simulink model "SWC_HALOUT_type"  (R2021b)
settings: Solver=FixedStepDiscrete  StartTime=0.0  StopTime=10.0  FixedStep=0.005  RelTol=1e-3
undefined symbols (not defined in the file): DIDLen_APPD, DIDLen_APPE, DIDLen_APPPedalZP, DIDLen_APSFunConfig, DIDLen_AutoLock, DIDLen_AutoWipHSpdEN, DIDLen_CALID, DIDLen_CDEODT, DIDLen_CLRDIST, DIDLen_DKCBLESta, DIDLen_DKCKey, DIDLen_DKCSta, DIDLen_DoorNFCAnchorSta, DIDLen_DRLDis, DIDLen_DynoMode, DIDLen_ECUNAME, DIDLen_FDDKCCoordXY, DIDLen_FMHTimer, DIDLen_LFLowPresThre, DIDLen_LFSensorID, DIDLen_LIDAAnchorSta, DIDLen_LRLowPresThre, DIDLen_LRSensorID, DIDLen_MILDIST, DIDLen_NUMPSATRIPSFLTMEMCLR, DIDLen_NVMPedalZP, DIDLen_OBDReq, DIDLen_ODOMETER, DIDLen_PKE, DIDLen_ProtocolId, DIDLen_PSA, DIDLen_QTYPSATRIPS, DIDLen_RFLowPresThre, DIDLen_RFSensorID, DIDLen_RRLowPresThre, DIDLen_RRSensorID, DIDLen_RUNTM, DIDLen_SensorMode, DIDLen_TestGroup, DIDLen_TireSize, DIDLen_TPMSLearnSta, DIDLen_TurnLampFLThreCurr, DIDLen_TurnLampFRThreCurr, DIDLen_TurnLampRLThreCurr, DIDLen_TurnLampRRThreCurr, DIDLen_UIDSta, DIDLen_USSConfig, DIDLen_UWBAnchorSta, DIDLen_VIN, DIDLen_VSS, DIDLen_WhlPres, DIDLen_WhlSensorBattSta, DIDLen_WhlTmp, DIDLen_WipRLSCmdCutFilter, DIDLen_WipRLSCmdHoldFilter, DIDLen_XWDMode, DIDNum_APPD, DIDNum_APPE, DIDNum_APPPedalZP, DIDNum_APSFunConfig ... (+504)
libraries: simulink x893, FVT_lib x320, hdlsllib x6, hcu_lib x5, halout x1
(part 10 of 11)

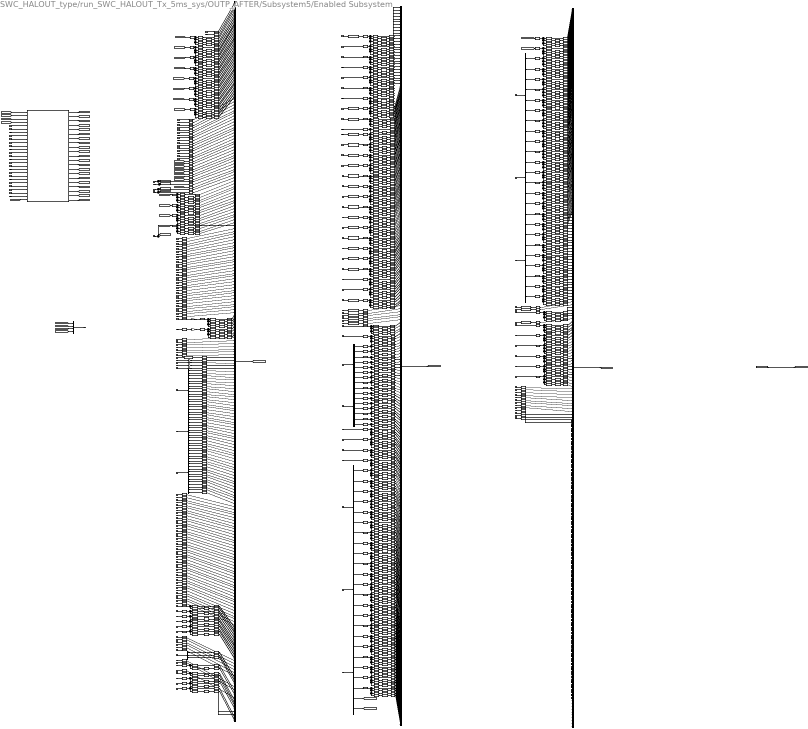
== system SWC_HALOUT_type/run_SWC_HALOUT_Tx_5ms_sys/OUTP_AFTER/Subsystem5/Enabled Subsystem ==
  VOUTP_AntitheftSta_enum : Inport
  VOUTP_DrivetrainSelect_enum : Inport  Port=2
  VOUTP_WriteChkLFID_raw : Inport  Port=3
  VOUTP_WriteChkRFID_raw : Inport  Port=4
  VOUTP_WriteChkLRID_raw : Inport  Port=5
  VOUTP_WriteChkRRID_raw : Inport  Port=6
  VOUTP_WriteChkfinLFID_raw : Inport  Port=7
  VOUTP_WriteChkfinRFID_raw : Inport  Port=8
  VOUTP_WriteChkfinLRID_raw : Inport  Port=9
  VOUTP_WriteChkfinRRID_raw : Inport  Port=10
  VOUTP_LFSensorFail_flg : Inport  Port=11
  VOUTP_RFSensorFail_flg : Inport  Port=12
  VOUTP_LRSensorFail_flg : Inport  Port=13
  VOUTP_RRSensorFail_flg : Inport  Port=14
  VOUTP_LFWheelPSW_raw8 : Inport  Port=15
  VOUTP_RFWheelPSW_raw8 : Inport  Port=16
  VOUTP_LRWheelPSW_raw8 : Inport  Port=17
  VOUTP_RRWheelPSW_raw8 : Inport  Port=18
  VOUTP_LFPindi_enum : Inport  Port=19
  VOUTP_RFPindi_enum : Inport  Port=20
  VOUTP_LRPindi_enum : Inport  Port=21
  VOUTP_RRPindi_enum : Inport  Port=22
  VOUTP_LFP20_raw8 : Inport  Port=23
  VOUTP_RFP20_raw8 : Inport  Port=24
  VOUTP_LRP20_raw8 : Inport  Port=25
  VOUTP_RRP20_raw8 : Inport  Port=26
  VOUTP_LFWheelPress_raw8 : Inport  Port=27
  VOUTP_RFWheelPress_raw8 : Inport  Port=28
  VOUTP_LRWheelPress_raw8 : Inport  Port=29
  VOUTP_RRWheelPress_raw8 : Inport  Port=30
  VOUTP_LFWheelTemp_C : Inport  Port=31
  VOUTP_RFWheelTemp_C : Inport  Port=32
  VOUTP_LRWheelTemp_C : Inport  Port=33
  VOUTP_RRWheelTemp_C : Inport  Port=34
  VOUTP_Flashchkdatavalid_enum : Inport  Port=35
  VOUTP_Flashdatavalid_enum : Inport  Port=36
  VOUTP_unlearnSfali_flg : Inport  Port=37
  VOUTP_unlearnSfailvalid_enum : Inport  Port=38
  VOUTP_Prepresstempvalid_enum : Inport  Port=39
  VOUTP_FlashS1ID_raw : Inport  Port=40
  VOUTP_FlashS2ID_raw : Inport  Port=41
  VOUTP_FlashS3ID_raw : Inport  Port=42
  VOUTP_FlashS41ID_raw : Inport  Port=43
  VOUTP_FlashIDvalid_enum : Inport  Port=44
  VOUTP_ACModeMem_enum : Inport  Port=45
  VOUTP_Face_flg : Inport  Port=46
  VOUTP_Foot_flg : Inport  Port=47
  VOUTP_Frost_flg : Inport  Port=48
  VOUTP_FaceM_flg : Inport  Port=49
  VOUTP_FootM_flg : Inport  Port=50
  VOUTP_CCUSyncSts_flg : Inport  Port=51
  VOUTP_ACForceOFF_flg : Inport  Port=52
  VOUTP_sigRecircSt_flg : Inport  Port=53
  VOUTP_RecAutoFlg_flg : Inport  Port=54
  VOUTP_AirIntenZone1M_enum : Inport  Port=55
  VOUTP_fdefog_flg : Inport  Port=56
  VOUTP_sigSetTempZon1St_C : Inport  Port=57
  VOUTP_sigSetTempZon2StM_C : Inport  Port=58
  VOUT_CountAlarm_enum : Inport  Port=59
  VOUTP_MFSWTri_flg : Inport  Port=60
  VOUTP_MirrorFlodPos_flg : Inport  Port=61
  VOUTP_FuelDoorPos_flg : Inport  Port=62
  VOUTP_LockSetting_flg : Inport  Port=63
  VOUTP_MFRDNBrightReq_pct : Inport  Port=64
  VOUTP_RoomLampMode_flg : Inport  Port=65
  VOUTP_WiperFixMode_flg : Inport  Port=66
  VOUTP_IVIPTGUSStaSW_flg : Inport  Port=67
  VOUTP_EAPS1MIN_pct : Inport  Port=68
  VOUTP_EAPS2MIN_pct : Inport  Port=69
  VOUTP_HoodSW_flg : Inport  Port=70
  VOUTP_TailgateSW_flg : Inport  Port=71
  VOUTP_CTDLockSW_flg : Inport  Port=72
  VOUTP_TailgateHDSW_flg : Inport  Port=73
  VOUTP_APMDoorControlSta_flg : Inport  Port=74
  VOUTP_fUnlockSingle_flg : Inport  Port=75
  VOUTP_SaveRegenMode_enum : Inport  Port=76
  VOUTP_AmbFunENFlash_enum : Inport  Port=77
  VOUTP_AmbWelENFlash_enum : Inport  Port=78
  VOUTP_AmbDimENFlash_enum : Inport  Port=79
  VOUTP_AmbLinkDriStaFlash_enum : Inport  Port=80
  VOUTP_AmbPwrWarnENFlash_enum : Inport  Port=81
  VOUTP_AmbODAENFlash_enum : Inport  Port=82
  VOUTP_AmbColorSta1_enum : Inport  Port=83
  VOUTP_AmbColorSta2_enum : Inport  Port=84
  VOUTP_AmbColorSta3_enum : Inport  Port=85
  VOUTP_AmbColorSta4_enum : Inport  Port=86
  VOUTP_AmbColorSta5_enum : Inport  Port=87
  VOUTP_AmbColorSta7_enum : Inport  Port=88
  VOUTP_AmbBrightnessSta1_enum : Inport  Port=89
  VOUTP_AmbBrightnessSta2_enum : Inport  Port=90
  VOUTP_AmbBrightnessSta3_enum : Inport  Port=91
  VOUTP_AmbBrightnessSta4_enum : Inport  Port=92
  VOUTP_AmbBrightnessSta5_enum : Inport  Port=93
  VOUTP_AmbBrightnessSta7_enum : Inport  Port=94
  VOUTP_TurnSwTimeSetSta123_enum : Inport  Port=95
  VOUTP_TurnSwTimeSetSta457_enum : Inport  Port=96
  VOUTP_FDCTHCAirIntZ3Sta_enum : Inport  Port=97
  VOUTP_FDCTHCREVentModeSta_enum : Inport  Port=98
  VOUTP_FDCTHCLEVentModeSta_enum : Inport  Port=99
  VOUTP_FDCTHCLEVentZSta_enum : Inport  Port=100
  VOUTP_FDCTHCCLEVentZSta_enum : Inport  Port=101
  VOUTP_FDCTHCREVentZSta_enum : Inport  Port=102
  VOUTP_FDCTHCCREVentZSta_enum : Inport  Port=103
  VOUTP_LVentEN_flg : Inport  Port=104
  VOUTP_FDCTHCLEVentYSta_enum : Inport  Port=105
  VOUTP_CLVentEN_flg : Inport  Port=106
  VOUTP_FDCTHCCLEVentYSta_enum : Inport  Port=107
  VOUTP_RVentEN_flg : Inport  Port=108
  VOUTP_FDCTHCREVentYSta_enum : Inport  Port=109
  VOUTP_CRVentEN_flg : Inport  Port=110
  VOUTP_FDCTHCCREVentYSta_enum : Inport  Port=111
  VOUTP_FDCFGSAirIntSta_enum : Inport  Port=112
  VOUTP_FDCFGSChSta_enum : Inport  Port=113
  VOUTP_FDCFGSIONSWSta_flg : Inport  Port=114
  VOUTP_WalkOutLkENFunSta_flg : Inport  Port=115
  VOUTP_WalkInUnLkENFunSta_flg : Inport  Port=116
  VOUTP_FollowMeENFunSta_flg : Inport  Port=117
  VOUTP_PTGUserHeight1_cnt : Inport  Port=118
  VOUTP_PTGUserHeight2_cnt : Inport  Port=119
  VOUTP_PTGUserHeight3_cnt : Inport  Port=120
  VOUTP_PTGUserHeight4_cnt : Inport  Port=121
  VOUTP_PTGUserHeight5_cnt : Inport  Port=122
  VOUTP_PTGUserHeight7_cnt : Inport  Port=123
  VOUTP_PTGOpenHeight12_enum : Inport  Port=124
  VOUTP_PTGOpenHeight34_enum : Inport  Port=125
  VOUTP_PTGOpenHeight57_enum : Inport  Port=126
  VOUTP_ACCLevelMem12_enum : Inport  Port=127
  VOUTP_ACCLevelMem34_enum : Inport  Port=128
  VOUTP_ACCLevelMem57_enum : Inport  Port=129
  VOUTP_AutoLockMem_enum : Inport  Port=130
  VOUTP_AutoUnlockMem_enum : Inport  Port=131
  VOUTP_MILDIST_km : Inport  Port=132
  VOUTP_CLRDIST_km : Inport  Port=133
  VOUTP_WARMUPS_cnt : Inport  Port=134
  VOUTP_MILTIME_min : Inport  Port=135
  VOUTP_CLRTIME_min : Inport  Port=136
  VOUTP_NUMPSATRIPSFLTMEMCLR_cnt : Inport  Port=137
  VOUTP_PSAR_sec : Inport  Port=138
  VOUTP_PSAL_sec : Inport  Port=139
  VOUTP_IPSAR_sec : Inport  Port=140
  VOUTP_IPSAL_sec : Inport  Port=141
  VOUTP_CPSAR_sec : Inport  Port=142
  VOUTP_CPSAL_sec : Inport  Port=143
  VOUTP_HVBNAH_Ahr : Inport  Port=144
  VOUTP_IGNCNTR_cnt : Inport  Port=145
  VOUTP_TNBCPSAR_Ahr : Inport  Port=146
  VOUTP_TNBCPSAL_Ahr : Inport  Port=147
  VOUTP_TNECPSAR_kWh : Inport  Port=148
  VOUTP_TNECPSAL_kWh : Inport  Port=149
  VOUTP_TEBPSAR_kWh : Inport  Port=150
  VOUTP_TEBPSAL_kWh : Inport  Port=151
  VOUTP_TGEOVCR_kWh : Inport  Port=152
  VOUTP_TGEOVCL_kWh : Inport  Port=153
  VOUTP_GECHGOVCDCR_kWh : Inport  Port=154
  VOUTP_GECHGOVCDCL_kWh : Inport  Port=155
  VOUTP_GECHGOVCACR_kWh : Inport  Port=156
  VOUTP_GECHGOVCACL_kWh : Inport  Port=157
  VOUTP_RESSV2XENNONPSAR_kWh : Inport  Port=158
  VOUTP_RESSV2XENNONPSAL_kWh : Inport  Port=159
  VOUTP_PKERNumerator_kphsqr : Inport  Port=160
  VOUTP_PKELNumerator_kphsqr : Inport  Port=161
  VOUTP_ODOMETER_km : Inport  Port=162
  VOUTP_ResetCDEODTR_km : Inport  Port=163
  VOUTP_AvgBattTempPSAR_C : Inport  Port=164
  VOUTP_AvgBattTempPSAL_C : Inport  Port=165
  VOUTP_AvgBattTempOVCR_C : Inport  Port=166
  VOUTP_AvgBattTempOVCL_C : Inport  Port=167
  VOUTP_AvgBattTempOFFR_C : Inport  Port=168
  VOUTP_AvgBattTempOFFL_C : Inport  Port=169
  VOUTP_HVBNE_kWh : Inport  Port=170
  VOUTP_QTYPSATRIPSR_cnt : Inport  Port=171
  VOUTP_QTYPSATRIPSL_cnt : Inport  Port=172
  VOUTP_RESSCNTDODRNGR_cnt : Inport  Port=173
  VOUTP_ETMBTOER_kWh : Inport  Port=174
  VOUTP_ETMBTOEL_kWh : Inport  Port=175
  VOUTP_RESSCNTDODRNGL_cnt : Inport  Port=176
  VOUTP_ETMATOER_kWh : Inport  Port=177
  VOUTP_ETMATOEL_kWh : Inport  Port=178
  VOUTP_RESSTIMESOCPSARNGR_s : Inport  Port=179
  VOUTP_RESSTIMESOCPSARNGL_s : Inport  Port=180
  VOUTP_RESSTIMESOCCHGRNGR_s : Inport  Port=181
  VOUTP_RESSTIMESOCOFFRNGL_s : Inport  Port=182
  VOUTP_MAXBATTEMPL_C : Inport  Port=183
  VOUTP_MINBATTEMPL_C : Inport  Port=184
  VOUTP_RESSTIMESOCCHGRNGL_s : Inport  Port=185
  VOUTP_RESSTIMESOCOFFRNGR_s : Inport  Port=186
  VOUTP_AVGBATTEMPL_sec : Inport  Port=187
  VOUTP_AVGBATTEMPL_C : Inport  Port=188
  VOUTP_BattTempPSAR_sec : Inport  Port=189
  VOUTP_BattTempPSAL_sec : Inport  Port=190
  VOUTP_OVCR_sec : Inport  Port=191
  VOUTP_OVCL_sec : Inport  Port=192
  VOUTP_OFFR_sec : Inport  Port=193
  VOUTP_OFFL_sec : Inport  Port=194
  VOUTP_HMIKey1FuncSta_enum : Inport  Port=195
  VOUTP_HMIKey2FuncSta_enum : Inport  Port=196
  VOUTP_HMIKey3FuncSta_enum : Inport  Port=197
  VOUTP_HMIKey4FuncSta_enum : Inport  Port=198
  VOUTP_HMIKey5FuncSta_enum : Inport  Port=199
  VOUTP_HMIKey6FuncSta_enum : Inport  Port=200
  VOUTP_HMIKey7FuncSta_enum : Inport  Port=201
  VOUTP_HMIKey8FuncSta_enum : Inport  Port=202
  VOUTP_AutoWipHSpdENSta_flg : Inport  Port=203
  VOUTP_ModelVersion_raw : Inport  Port=204
  VOUTP_ModelVersionChksum_raw : Inport  Port=205
  VOUTP_DIDModelVersion_raw : Inport  Port=206
  VOUTP_DIDModelVersionChksum_raw : Inport  Port=207
  BHAL_SYS_outputs : Inport  Port=208
  VHAL_RandomnumberY_raw1 : Inport  Port=209
  VHAL_RandomnumberY_raw2 : Inport  Port=210
  VHAL_RandomnumberY_raw3 : Inport  Port=211
  VHAL_RandomnumberY_raw4 : Inport  Port=212
  VHAL_RandomnumberY_raw5 : Inport  Port=213
  VHAL_RandomnumberY_raw6 : Inport  Port=214
  VHAL_RandomnumberY_raw7 : Inport  Port=215
  VHAL_RandomnumberY_raw8 : Inport  Port=216
  VHAL_funAuto_flg : Inport  Port=217
  VHAL_DiagDRLOFF_flg : Inport  Port=218
  VHAL_DiagFMHT_s : Inport  Port=219
  VHAL_DiagFLTC_mA : Inport  Port=220
  VHAL_DiagFRTC_mA : Inport  Port=221
  VHAL_DiagRLTC_mA : Inport  Port=222
  VHAL_DiagRRTC_mA : Inport  Port=223
  VHAL_USSConfig_raw8 : Inport  Port=224
  VHAL_TireSize_raw8 : Inport  Port=225
  VHAL_APSFunConfig_raw8 : Inport  Port=226
  BHAL_DIDGetData_raw : Inport  Port=227
  Bitwise AND{,4,8,14,16,22,26,30,32,36,40,44,48,52,56,58,60,62,64,66,68,70,72,74,76,80,82,86,90,94,98,102,106,110,114,116,120,124,128,132,136,140,144,148,152,156,160,164,168,172,176,180,184,188,192,194,196,198,200,202,204,206,208,210,212,214,216,218,220,222,224,228,232,236,240,244,248,252,256,260,264,268,272,276,280,284,288,292,296,300,304,308,312,316,320,324,328,332,336,340,344,348,352,356,360,364,368,372,376,380,384,388,392,396,400,404,408,412,416,420,424,428,432,436,440,444,448,452,456} (129 alike) : simulink/Logic and Bit Operations/Bitwise Operator  logicop=AND  UseBitMask=on  BitMask=bin2dec('00000000000000000000000011111111')  BitMaskRealWorld=Stored Integer
  Bitwise AND{1,5,9,15,17,23,27,31,33,37,41,45,49,53,57,59,61,63,65,67,69,71,73,75,77,81,83,87,91,95,99,103,107,111,115,117,121,125,129,133,137,141,145,149,153,157,161,165,169,173,177,181,185,189,193,195,197,199,201,203,205,207,209,211,213,215,217,219,221,223,225,229,233,237,241,245,249,253,257,261,265,269,273,277,281,285,289,293,297,301,305,309,313,317,321,325,329,333,337,341,345,349,353,357,361,365,369,373,377,381,385,389,393,397,401,405,409,413,417,421,425,429,433,437,441,445,449,453,457} (129 alike) : simulink/Logic and Bit Operations/Bitwise Operator  logicop=AND  UseBitMask=on  BitMask=bin2dec('00000000000000001111111100000000')  BitMaskRealWorld=Stored Integer
  Bitwise AND{2,6,10,12,18,20,24,28,34,38,42,46,50,54,78,84,88,92,96,100,104,108,112,118,122,126,130,134,138,142,146,150,154,158,162,166,170,174,178,182,186,190,226,230,234,238,242,246,250,254,258,262,266,270,274,278,282,286,290,294,298,302,306,310,314,318,322,326,330,334,338,342,346,350,354,358,362,366,370,374,378,382,386,390,394,398,402,406,410,414,418,422,426,430,434,438,442,446,450,454,458} (101 alike) : simulink/Logic and Bit Operations/Bitwise Operator  logicop=AND  UseBitMask=on  BitMask=bin2dec('00000000111111110000000000000000')  BitMaskRealWorld=Stored Integer
  Bitwise AND{3,7,11,13,19,21,25,29,35,39,43,47,51,55,79,85,89,93,97,101,105,109,113,119,123,127,131,135,139,143,147,151,155,159,163,167,171,175,179,183,187,191,227,231,235,239,243,247,251,255,259,263,267,271,275,279,283,287,291,295,299,303,307,311,315,319,323,327,331,335,339,343,347,351,355,359,363,367,371,375,379,383,387,391,395,399,403,407,411,415,419,423,427,431,435,439,443,447,451,455,459} (101 alike) : simulink/Logic and Bit Operations/Bitwise Operator  logicop=AND  UseBitMask=on  BitMask=bin2dec('11111111000000000000000000000000')  BitMaskRealWorld=Stored Integer
  Bus Selector2 : BusSelector  OutputSignals=VHAL_AutoWipHSpdEN_raw,VHAL_WipRLSCmdHoldFilter_raw,VHAL_WipRLSCmdCutFilter_raw
  Constant : Constant  Value=zeros(256,1)  OutDataTypeStr=uint8
  Data Type Conversion{,1,5..13,15..18,20..23,25..27,29..32,34..37,39..40,42..106,108..111,113..116,118..121,123..126,128..130,132..235,237..239,241..242,244..245,247..248,250..251,253..265,267..269,271..272,274..275,277..278,280..283,285..286,288..291,293..296,298..301,303..306,308..311,313..316,318..321,323..326,328..329,331..334,336..339,341..344,346..349,351..354,356..359,361..364,366..369,371..374,376..379,381..384,386..389,391..394,396..399,401..404,406..415,417..420,422..425,427..430,432..433,435..436,438..439,441..442,444..445,447..448,450..451,453..454,456..457,459..460,462..463,465..466,468..469,471..472,474..475,477..478,480..483,485..488,490..493,495..498,500..503,505..508,510..513,515..518,520..523,525..528,530..533,535..538,540..543,545..548,550..553,555..558,560..563,565..568,570..573,575..578,580..583,585..588,590..593,595..598,600..603,605..608,610..613,615..618,620..623,625..628,630..633,635..638,640..643,645..648,650..653,655..658,660..663,665..668,670..673,675..678,680..683,685..688,690..693,695..698,700..703,705..708,710..713,715..718,720..723,725..728,730..733,735..740,742..746,748..751,753..756,758..761,763..766,768..771,773..789} (659 alike) : DataTypeConversion  OutDataTypeStr=uint8
  Data Type Conversion{4,14,19,24,28,33,38,41,107,112,117,122,127,131,279,287,292,297,302,307,312,317,322,330,335,340,345,350,355,360,365,370,375,380,385,390,395,400,405,416,421,426,479,484,489,494,499,504,509,514,519,524,529,534,539,544,549,554,559,564,569,574,579,584,589,594,599,604,609,614,619,624,629,634,639,644,649,654,659,664,669,674,679,684,689,694,699,704,709,714,719,724,729,734,741,747,752,757,762,767,772} (101 alike) : DataTypeConversion  OutDataTypeStr=uint32
  Data Type Conversion2 : DataTypeConversion  OutDataTypeStr=single
  Data Type Conversion{236,240,243,246,249,252,266,270,273,276,284,327,431,434,437,440,443,446,449,452,455,458,461,464,467,470,473,476} (28 alike) : DataTypeConversion  OutDataTypeStr=uint16
  Data Type Conversion3 : DataTypeConversion  OutDataTypeStr=single
  Demux : Demux  Outputs=16
  Demux1 : Demux  Outputs=16
  Demux{3..10} (8 alike) : Demux  Outputs=8
  Demux2 : Demux  Outputs=16
  Gain{,1..3} (4 alike) : Gain  Gain=1/10
  Ground_{14..121} (108 alike) : Ground
  Multiply : Gain  Gain=10000
  Multiply1 : Gain  Gain=10000
  Mux : Mux  Inputs=256
  Mux1 : Mux  Inputs=256
  Mux2 : Mux
  Mux3 : Mux  Inputs=256
  NVM1 : Subsystem
  Shift Arithmetic{,3,6,9,12,17,20,23..24,27,30,33,36,39,42..52,55..56,59,62,65,68,71,74,77,80..81,84,87,90,93,96,99,104,107,110,113,116,119,122,125,128,131,134,137..153,156,159,162,165,168,171,174,177,180,183,186,189,192,195,198,201,204,207,210,213,216,219,222,225,228,231,234,237,240,243,246,249,252,255,258,261,264,267,270,273,276,279,282,285,288,291,294,297,300,303,306,309,312,315,318,321,324,327,330} (129 alike) : ArithShift  BitShiftNumber=8  BitShiftDirection=Right
  Shift Arithmetic{1,4,7,10,13..14,18,21,25,28,31,34,37,40,53,57,60,63,66,69,72,75,78,82,85,88,91,94,97,100,102,105,108,111,114,117,120,123,126,129,132,135,154,157,160,163,166,169,172,175,178,181,184,187,190,193,196,199,202,205,208,211,214,217,220,223,226,229,232,235,238,241,244,247,250,253,256,259,262,265,268,271,274,277,280,283,286,289,292,295,298,301,304,307,310,313,316,319,322,325,328} (101 alike) : ArithShift  BitShiftNumber=16  BitShiftDirection=Right
  Shift Arithmetic{2,5,8,11,15..16,19,22,26,29,32,35,38,41,54,58,61,64,67,70,73,76,79,83,86,89,92,95,98,101,103,106,109,112,115,118,121,124,127,130,133,136,155,158,161,164,167,170,173,176,179,182,185,188,191,194,197,200,203,206,209,212,215,218,221,224,227,230,233,236,239,242,245,248,251,254,257,260,263,266,269,272,275,278,281,284,287,290,293,296,299,302,305,308,311,314,317,320,323,326,329} (101 alike) : ArithShift  BitShiftNumber=24  BitShiftDirection=Right
  Subsystem : Subsystem
  convert_in{,5..16,23} (14 alike) : FVT_lib/hal/convert_in  gain=10  offset=0
  convert_in1 : FVT_lib/hal/convert_in  gain=1000  offset=2147483648
  convert_in{17..22,24..26} (9 alike) : FVT_lib/hal/convert_in  gain=1  offset=40
  convert_in2 : FVT_lib/hal/convert_in  gain=1000  offset=2147483648
  convert_in3 : FVT_lib/hal/convert_in  gain=1000  offset=0
  convert_in4 : FVT_lib/hal/convert_in  gain=1000  offset=0
  HAL_NvmWriteData_raw : Outport
  wires:
  Bitwise AND20/1 -> Shift Arithmetic14/1
  Shift Arithmetic4/1 -> Data Type Conversion12/1
  Data Type Conversion12/1 -> Mux/9
  Data Type Conversion30/1 -> Mux/24
  Shift Arithmetic23/1 -> Data Type Conversion40/1
  Bitwise AND1/1 -> Shift Arithmetic/1
  Bitwise AND11/1 -> Shift Arithmetic8/1
  Data Type Conversion5/1 -> Mux/21
  Bitwise AND17/1 -> Shift Arithmetic12/1
  Data Type Conversion32/1 -> Mux/30
  Data Type Conversion13/1 -> Mux/10
  Shift Arithmetic22/1 -> Data Type Conversion32/1
  Shift Arithmetic17/1 -> Data Type Conversion30/1
  Shift Arithmetic18/1 -> Data Type Conversion7/1
  Data Type Conversion14/1 -> Bitwise AND4/1, Bitwise AND7/1, Bitwise AND6/1, Bitwise AND5/1
  Bitwise AND26/1 -> Data Type Conversion29/1
  Data Type Conversion17/1 -> Mux/13
  Data Type Conversion25/1 -> Mux/15
  Data Type Conversion18/1 -> Mux/14
  Bitwise AND29/1 -> Shift Arithmetic19/1
  Shift Arithmetic8/1 -> Data Type Conversion18/1
  Data Type Conversion39/1 -> Mux/31
  Shift Arithmetic10/1 -> Data Type Conversion22/1
  Data Type Conversion6/1 -> Mux/22
  Bitwise AND28/1 -> Shift Arithmetic18/1
  Shift Arithmetic/1 -> Data Type Conversion9/1
  Data Type Conversion42/1 -> Mux/19
  Data Type Conversion11/1 -> Mux/6
  Shift Arithmetic19/1 -> Data Type Conversion27/1
  Data Type Conversion28/1 -> Bitwise AND26/1, Bitwise AND27/1, Bitwise AND28/1, Bitwise AND29/1
  Bitwise AND19/1 -> Shift Arithmetic22/1
  Bitwise AND27/1 -> Shift Arithmetic17/1
  Bitwise AND3/1 -> Shift Arithmetic2/1
  Data Type Conversion1/1 -> Mux/2
  Data Type Conversion26/1 -> Mux/16
  Bitwise AND23/1 -> Shift Arithmetic23/1
  Shift Arithmetic7/1 -> Data Type Conversion17/1
  Shift Arithmetic21/1 -> Data Type Conversion31/1
  Data Type Conversion8/1 -> Mux/3
  Data Type Conversion/1 -> Mux/1
  Bitwise AND10/1 -> Shift Arithmetic7/1
  Data Type Conversion37/1 -> Mux/34
  Data Type Conversion40/1 -> Mux/32
  Data Type Conversion36/1 -> Mux/33
  Bitwise AND/1 -> Data Type Conversion8/1
  Data Type Conversion20/1 -> Mux/11
  Data Type Conversion16/1 -> Mux/8
  Data Type Conversion21/1 -> Mux/12
  Data Type Conversion9/1 -> Mux/4
  Data Type Conversion10/1 -> Mux/5
  Data Type Conversion31/1 -> Mux/29
  Data Type Conversion15/1 -> Mux/7
  Data Type Conversion34/1 -> Mux/27
  Data Type Conversion35/1 -> Mux/28
  Data Type Conversion27/1 -> Mux/26
  Data Type Conversion29/1 -> Mux/23
  Data Type Conversion7/1 -> Mux/25
  Data Type Conversion22/1 -> Mux/17
  Data Type Conversion23/1 -> Mux/18
  Data Type Conversion43/1 -> Mux/20
  Data Type Conversion33/1 -> Bitwise AND19/1, Bitwise AND18/1, Bitwise AND31/1, Bitwise AND30/1
  Data Type Conversion41/1 -> Bitwise AND25/1, Bitwise AND24/1, Bitwise AND17/1, Bitwise AND16/1
  Bitwise AND30/1 -> Data Type Conversion34/1
  Bitwise AND24/1 -> Shift Arithmetic13/1
  Shift Arithmetic12/1 -> Data Type Conversion43/1
  Bitwise AND25/1 -> Shift Arithmetic16/1
  Bitwise AND18/1 -> Shift Arithmetic21/1
  Shift Arithmetic16/1 -> Data Type Conversion6/1
  Shift Arithmetic15/1 -> Data Type Conversion37/1
  Data Type Conversion38/1 -> Bitwise AND21/1, Bitwise AND20/1, Bitwise AND23/1, Bitwise AND22/1
  Bitwise AND31/1 -> Shift Arithmetic20/1
  Shift Arithmetic9/1 -> Data Type Conversion26/1
  Bitwise AND21/1 -> Shift Arithmetic15/1
  Data Type Conversion24/1 -> Bitwise AND14/1, Bitwise AND13/1, Bitwise AND12/1, Bitwise AND15/1
  Bitwise AND13/1 -> Shift Arithmetic11/1
  Bitwise AND9/1 -> Shift Arithmetic6/1
  Bitwise AND15/1 -> Shift Arithmetic9/1
  Bitwise AND12/1 -> Shift Arithmetic10/1
  Bitwise AND7/1 -> Shift Arithmetic5/1
  Shift Arithmetic2/1 -> Data Type Conversion11/1
  Shift Arithmetic1/1 -> Data Type Conversion10/1
  Data Type Conversion19/1 -> Bitwise AND11/1, Bitwise AND10/1, Bitwise AND9/1, Bitwise AND8/1
  Bitwise AND6/1 -> Shift Arithmetic4/1
  Bitwise AND5/1 -> Shift Arithmetic3/1
  Shift Arithmetic20/1 -> Data Type Conversion35/1
  Shift Arithmetic5/1 -> Data Type Conversion13/1
  Bitwise AND4/1 -> Data Type Conversion15/1
  Shift Arithmetic3/1 -> Data Type Conversion16/1
  Bitwise AND8/1 -> Data Type Conversion20/1
  Bitwise AND22/1 -> Data Type Conversion39/1
  Data Type Conversion4/1 -> Bitwise AND3/1, Bitwise AND2/1, Bitwise AND1/1, Bitwise AND/1
  Bitwise AND2/1 -> Shift Arithmetic1/1
  Shift Arithmetic11/1 -> Data Type Conversion23/1
  Shift Arithmetic14/1 -> Data Type Conversion36/1
  Shift Arithmetic13/1 -> Data Type Conversion5/1
  Bitwise AND14/1 -> Data Type Conversion25/1
  Shift Arithmetic6/1 -> Data Type Conversion21/1
  Bitwise AND16/1 -> Data Type Conversion42/1
  VOUTP_DrivetrainSelect_enum/1 -> Data Type Conversion1/1
  VOUTP_AntitheftSta_enum/1 -> Data Type Conversion/1
  Data Type Conversion66/1 -> Mux/57
  Data Type Conversion67/1 -> Mux/55
  VOUTP_ACModeMem_enum/1 -> Data Type Conversion81/1
  Data Type Conversion57/1 -> Mux/48
  VHAL_RandomnumberY_raw7/1 -> Data Type Conversion79/1
  VHAL_RandomnumberY_raw5/1 -> Data Type Conversion77/1
  VHAL_RandomnumberY_raw6/1 -> Data Type Conversion78/1
  Data Type Conversion72/1 -> Mux/62
  Data Type Conversion69/1 -> Mux/59
  VOUTP_Foot_flg/1 -> Data Type Conversion83/1
  [VHAL_NVMLRWheelPress_raw8] -> Data Type Conversion62/1
  VOUTP_LFSensorFail_flg/1 -> Data Type Conversion47/1
  [VHAL_NVMLFWheelPress_raw8] -> Data Type Conversion63/1
  VHAL_RandomnumberY_raw4/1 -> Data Type Conversion76/1
  VOUTP_Flashchkdatavalid_enum/1 -> [VOUTP_Flashchkdatavalid_enum], Data Type Conversion69/1
  Data Type Conversion63/1 -> Mux/51
  Data Type Conversion68/1 -> Mux/58
  Data Type Conversion51/1 -> Mux/39
  Data Type Conversion53/1 -> Mux/44
  VHAL_RandomnumberY_raw1/1 -> Data Type Conversion75/1
  Data Type Conversion48/1 -> Mux/38
  VOUTP_Face_flg/1 -> Data Type Conversion82/1
  VOUTP_LFP20_raw8/1 -> Data Type Conversion59/1
  VOUTP_CCUSyncSts_flg/1 -> Data Type Conversion87/1
  VHAL_RandomnumberY_raw3/1 -> Data Type Conversion74/1
  [VHAL_NVMRFWheelPress_raw8] -> Data Type Conversion61/1
  Data Type Conversion54/1 -> Mux/45
  Data Type Conversion47/1 -> Mux/35
  [VHAL_NVMunlearnSfali_flg] -> Data Type Conversion71/1
  VOUTP_RecAutoFlg_flg/1 -> Data Type Conversion90/1
  Data Type Conversion61/1 -> Mux/52
  VOUTP_fdefog_flg/1 -> Data Type Conversion92/1
  Data Type Conversion55/1 -> Mux/43
  VOUTP_sigRecircSt_flg/1 -> Data Type Conversion89/1
  Data Type Conversion52/1 -> Mux/42
  Data Type Conversion93/1 -> Mux/63
  Data Type Conversion56/1 -> Mux/46
  VOUTP_RFP20_raw8/1 -> Data Type Conversion57/1
  VOUTP_Prepresstempvalid_enum/1 -> [VOUTP_Prepresstempvalid_enum], Data Type Conversion93/1
  VOUTP_FaceM_flg/1 -> Data Type Conversion85/1
  Data Type Conversion58/1 -> Mux/49
  Data Type Conversion65/1 -> Mux/56
  VOUTP_RRPindi_enum/1 -> Data Type Conversion56/1
  VOUTP_FootM_flg/1 -> Data Type Conversion86/1
  Data Type Conversion50/1 -> Mux/41
  VOUTP_Flashdatavalid_enum/1 -> [VOUTP_Flashdatavalid_enum], Data Type Conversion70/1
  [VHAL_NVMRRWheelPress_raw8] -> Data Type Conversion64/1
  Data Type Conversion70/1 -> Mux/60
  [VHAL_NVMRRWheelTemp_C] -> Data Type Conversion68/1
  [VHAL_NVMLFWheelTemp_C] -> Data Type Conversion67/1
  VOUTP_AirIntenZone1M_enum/1 -> Data Type Conversion91/1
  Data Type Conversion64/1 -> Mux/54
  VOUTP_LRP20_raw8/1 -> Data Type Conversion58/1
  Data Type Conversion71/1 -> Mux/61
  VOUTP_RFPindi_enum/1 -> Data Type Conversion53/1
  VOUTP_RRP20_raw8/1 -> Data Type Conversion60/1
  Data Type Conversion49/1 -> Mux/40
  VOUTP_LRPindi_enum/1 -> Data Type Conversion54/1
  VOUTP_LFPindi_enum/1 -> Data Type Conversion55/1
  [VHAL_NVMLRWheelTemp_C] -> Data Type Conversion66/1
  Data Type Conversion62/1 -> Mux/53
  Data Type Conversion60/1 -> Mux/50
  Data Type Conversion59/1 -> Mux/47
  VOUTP_RRWheelPSW_raw8/1 -> Data Type Conversion52/1
  VHAL_RandomnumberY_raw2/1 -> Data Type Conversion73/1
  VOUTP_LRWheelPSW_raw8/1 -> Data Type Conversion50/1
  VHAL_RandomnumberY_raw8/1 -> Data Type Conversion80/1
  Data Type Conversion45/1 -> Mux/36
  VOUTP_ACForceOFF_flg/1 -> Data Type Conversion88/1
  Data Type Conversion46/1 -> Mux/37
  VOUTP_LFWheelPSW_raw8/1 -> Data Type Conversion51/1
  VOUTP_RRSensorFail_flg/1 -> Data Type Conversion48/1
  VOUTP_LRSensorFail_flg/1 -> Data Type Conversion46/1
  [VHAL_NVMRFWheelTemp_C] -> Data Type Conversion65/1
  VOUTP_RFWheelPSW_raw8/1 -> Data Type Conversion49/1
  VOUTP_RFSensorFail_flg/1 -> Data Type Conversion45/1
  VOUTP_Frost_flg/1 -> Data Type Conversion84/1
  Data Type Conversion134/1 -> Mux/120
  Data Type Conversion135/1 -> Mux/121
  Data Type Conversion136/1 -> Mux/122
  Data Type Conversion137/1 -> Mux/123
  Data Type Conversion255/1 -> Mux/235
  NVM1/1(VHAL_NVMWriteChkLFID_raw) -> [VHAL_NVMWriteChkLFID_raw]
  VOUTP_WriteChkRFID_raw/1 -> NVM1/6(VOUTP_WriteChkRFID_raw)
  VOUTP_WriteChkLFID_raw/1 -> NVM1/5(VOUTP_WriteChkLFID_raw)
  VOUTP_WriteChkRRID_raw/1 -> NVM1/8(VOUTP_WriteChkRRID_raw)
  VOUTP_WriteChkLRID_raw/1 -> NVM1/7(VOUTP_WriteChkLRID_raw)
  [VOUTP_unlearnSfailvalid_enum] -> NVM1/3(VOUTP_unlearnSfailvalid_enum)
  [VOUTP_Flashchkdatavalid_enum] -> NVM1/1(VOUTP_Flashchkdatavalid_enum)
  [VOUTP_Prepresstempvalid_enum] -> NVM1/4(VOUTP_Prepresstempvalid_enum)
  [VOUTP_Flashdatavalid_enum] -> NVM1/2(VOUTP_Flashdatavalid_enum)
  VOUTP_unlearnSfailvalid_enum/1 -> Data Type Conversion72/1, [VOUTP_unlearnSfailvalid_enum]
  [VHAL_NVMWriteChkfinRRID_raw] -> Data Type Conversion38/1
  [VHAL_NVMWriteChkfinLRID_raw] -> Data Type Conversion33/1
  [VHAL_NVMWriteChkfinRFID_raw] -> Data Type Conversion28/1
  [VHAL_NVMWriteChkfinLFID_raw] -> Data Type Conversion41/1
  [VHAL_NVMWriteChkRRID_raw] -> Data Type Conversion24/1
  [VHAL_NVMWriteChkLRID_raw] -> Data Type Conversion19/1
  [VHAL_NVMWriteChkRFID_raw] -> Data Type Conversion14/1
  [VHAL_NVMWriteChkLFID_raw] -> Data Type Conversion4/1
  VOUT_CountAlarm_enum/1 -> Data Type Conversion99/1
  VOUTP_FuelDoorPos_flg/1 -> Data Type Conversion96/1
  VOUTP_LockSetting_flg/1 -> Data Type Conversion103/1
  VOUTP_WiperFixMode_flg/1 -> Data Type Conversion104/1
  VOUTP_MFRDNBrightReq_pct/1 -> Data Type Conversion100/1
  VOUTP_IVIPTGUSStaSW_flg/1 -> Data Type Conversion102/1
  VOUTP_RoomLampMode_flg/1 -> Data Type Conversion101/1
  VOUTP_MirrorFlodPos_flg/1 -> Data Type Conversion95/1
  VOUTP_sigSetTempZon2StM_C/1 -> Data Type Conversion98/1
  VOUTP_sigSetTempZon1St_C/1 -> Data Type Conversion97/1
  VOUTP_MFSWTri_flg/1 -> Data Type Conversion94/1
  VOUTP_WriteChkfinLRID_raw/1 -> NVM1/11(VOUTP_WriteChkfinLRID_raw)
  VOUTP_WriteChkfinRRID_raw/1 -> NVM1/12(VOUTP_WriteChkfinRRID_raw)
  VOUTP_WriteChkfinLFID_raw/1 -> NVM1/9(VOUTP_WriteChkfinLFID_raw)
  VOUTP_WriteChkfinRFID_raw/1 -> NVM1/10(VOUTP_WriteChkfinRFID_raw)
  VOUTP_LFWheelPress_raw8/1 -> NVM1/13(VOUTP_LFWheelPress_raw8)
  VOUTP_RFWheelPress_raw8/1 -> NVM1/14(VOUTP_RFWheelPress_raw8)
  VOUTP_RRWheelPress_raw8/1 -> NVM1/16(VOUTP_RRWheelPress_raw8)
  VOUTP_LRWheelPress_raw8/1 -> NVM1/15(VOUTP_LRWheelPress_raw8)
  VOUTP_LFWheelTemp_C/1 -> NVM1/17(VOUTP_LFWheelTemp_C)
  VOUTP_RFWheelTemp_C/1 -> NVM1/18(VOUTP_RFWheelTemp_C)
  VOUTP_LRWheelTemp_C/1 -> NVM1/19(VOUTP_LRWheelTemp_C)
  VOUTP_RRWheelTemp_C/1 -> NVM1/20(VOUTP_RRWheelTemp_C)
  VOUTP_unlearnSfali_flg/1 -> NVM1/21(VOUTP_unlearnSfali_flg)
  BHAL_SYS_outputs/1 -> NVM1/22(BHAL_SYS_outputs)
  VOUTP_FlashS41ID_raw/1 -> NVM1/26(VOUTP_FlashS4ID_raw)
  VOUTP_FlashS2ID_raw/1 -> NVM1/24(VOUTP_FlashS2ID_raw)
  VOUTP_FlashS1ID_raw/1 -> NVM1/23(VOUTP_FlashS1ID_raw)
  VOUTP_FlashS3ID_raw/1 -> NVM1/25(VOUTP_FlashS3ID_raw)
  [VOUTP_FlashIDvalid_enum] -> NVM1/27(VOUTP_FlashIDvalid_enum)
  VOUTP_FlashIDvalid_enum/1 -> Mux/80, [VOUTP_FlashIDvalid_enum]
  Shift Arithmetic32/1 -> Data Type Conversion116/1
  Bitwise AND35/1 -> Shift Arithmetic26/1
  Shift Arithmetic29/1 -> Data Type Conversion111/1
  Bitwise AND43/1 -> Shift Arithmetic32/1
  Bitwise AND33/1 -> Shift Arithmetic24/1
  Bitwise AND41/1 -> Shift Arithmetic30/1
  [VHAL_NVMFlashS4ID_raw] -> Data Type Conversion122/1
  Shift Arithmetic24/1 -> Data Type Conversion109/1
  Data Type Conversion107/1 -> Bitwise AND35/1, Bitwise AND34/1, Bitwise AND33/1, Bitwise AND32/1
  Shift Arithmetic33/1 -> Data Type Conversion124/1
  Shift Arithmetic34/1 -> Data Type Conversion120/1
  Data Type Conversion117/1 -> Bitwise AND43/1, Bitwise AND42/1, Bitwise AND41/1, Bitwise AND40/1
  Bitwise AND36/1 -> Data Type Conversion113/1
  Bitwise AND40/1 -> Data Type Conversion118/1
  Shift Arithmetic27/1 -> Data Type Conversion114/1
  Bitwise AND32/1 -> Data Type Conversion108/1
  Bitwise AND37/1 -> Shift Arithmetic27/1
  Data Type Conversion122/1 -> Bitwise AND47/1, Bitwise AND46/1, Bitwise AND45/1, Bitwise AND44/1
  Shift Arithmetic26/1 -> Data Type Conversion106/1
  Data Type Conversion112/1 -> Bitwise AND39/1, Bitwise AND38/1, Bitwise AND37/1, Bitwise AND36/1
  Bitwise AND39/1 -> Shift Arithmetic29/1
  Bitwise AND47/1 -> Shift Arithmetic35/1
  Bitwise AND44/1 -> Data Type Conversion123/1
  Bitwise AND46/1 -> Shift Arithmetic34/1
  [VHAL_NVMFlashS3ID_raw] -> Data Type Conversion117/1
  Shift Arithmetic30/1 -> Data Type Conversion119/1
  Bitwise AND34/1 -> Shift Arithmetic25/1
  Shift Arithmetic28/1 -> Data Type Conversion110/1
  Bitwise AND38/1 -> Shift Arithmetic28/1
  Bitwise AND45/1 -> Shift Arithmetic33/1
  [VHAL_NVMFlashS2ID_raw] -> Data Type Conversion112/1
  Shift Arithmetic25/1 -> Data Type Conversion105/1
  Shift Arithmetic35/1 -> Data Type Conversion121/1
  Shift Arithmetic31/1 -> Data Type Conversion115/1
  Bitwise AND42/1 -> Shift Arithmetic31/1
  [VHAL_NVMFlashS1ID_raw] -> Data Type Conversion107/1
  Data Type Conversion109/1 -> Mux/65
  Data Type Conversion105/1 -> Mux/66
  Data Type Conversion106/1 -> Mux/67
  Data Type Conversion114/1 -> Mux/69
  Data Type Conversion110/1 -> Mux/70
  Data Type Conversion111/1 -> Mux/71
  Data Type Conversion119/1 -> Mux/73
  Data Type Conversion115/1 -> Mux/74
  Data Type Conversion116/1 -> Mux/75
  Data Type Conversion124/1 -> Mux/77
  Data Type Conversion120/1 -> Mux/78
  Data Type Conversion121/1 -> Mux/79
  Data Type Conversion108/1 -> Mux/64
  Data Type Conversion113/1 -> Mux/68
  Data Type Conversion118/1 -> Mux/72
  Data Type Conversion123/1 -> Mux/76
  Data Type Conversion75/1 -> Mux/81
  Data Type Conversion73/1 -> Mux/82
  Data Type Conversion74/1 -> Mux/83
  Data Type Conversion76/1 -> Mux/84
  Data Type Conversion77/1 -> Mux/85
  Data Type Conversion78/1 -> Mux/86
  Data Type Conversion79/1 -> Mux/87
  Data Type Conversion80/1 -> Mux/88
  Data Type Conversion81/1 -> Mux/89
  Data Type Conversion82/1 -> Mux/90
  Data Type Conversion83/1 -> Mux/91
  Data Type Conversion84/1 -> Mux/92
  Data Type Conversion85/1 -> Mux/93
  Data Type Conversion86/1 -> Mux/94
  Data Type Conversion87/1 -> Mux/95
  Data Type Conversion88/1 -> Mux/96
  Data Type Conversion89/1 -> Mux/97
  Data Type Conversion90/1 -> Mux/98
  Data Type Conversion91/1 -> Mux/99
  Data Type Conversion92/1 -> Mux/100
  Data Type Conversion97/1 -> Mux/101
  Data Type Conversion98/1 -> Mux/102
  Data Type Conversion99/1 -> Mux/103
  Data Type Conversion94/1 -> Mux/104
  Data Type Conversion95/1 -> Mux/105
  Data Type Conversion96/1 -> Mux/106
  Data Type Conversion103/1 -> Mux/107
  Data Type Conversion100/1 -> Mux/108
  Data Type Conversion101/1 -> Mux/109
  Data Type Conversion104/1 -> Mux/110
  Data Type Conversion102/1 -> Mux/111
  NVM1/21(VHAL_NVMFlashS4ID_raw) -> [VHAL_NVMFlashS4ID_raw]
  NVM1/2(VHAL_NVMWriteChkRFID_raw) -> [VHAL_NVMWriteChkRFID_raw]
  NVM1/3(VHAL_NVMWriteChkLRID_raw) -> [VHAL_NVMWriteChkLRID_raw]
  NVM1/4(VHAL_NVMWriteChkRRID_raw) -> [VHAL_NVMWriteChkRRID_raw]
  NVM1/5(VHAL_NVMWriteChkfinLFID_raw) -> [VHAL_NVMWriteChkfinLFID_raw]
  NVM1/6(VHAL_NVMWriteChkfinRFID_raw) -> [VHAL_NVMWriteChkfinRFID_raw]
  NVM1/7(VHAL_NVMWriteChkfinLRID_raw) -> [VHAL_NVMWriteChkfinLRID_raw]
  NVM1/8(VHAL_NVMWriteChkfinRRID_raw) -> [VHAL_NVMWriteChkfinRRID_raw]
  NVM1/9(VHAL_NVMunlearnSfali_flg) -> [VHAL_NVMunlearnSfali_flg]
  NVM1/10(VHAL_NVMLFWheelPress_raw8) -> [VHAL_NVMLFWheelPress_raw8]
  NVM1/11(VHAL_NVMRFWheelPress_raw8) -> [VHAL_NVMRFWheelPress_raw8]
  NVM1/12(VHAL_NVMLRWheelPress_raw8) -> [VHAL_NVMLRWheelPress_raw8]
  NVM1/13(VHAL_NVMRRWheelPress_raw8) -> [VHAL_NVMRRWheelPress_raw8]
  NVM1/14(VHAL_NVMLFWheelTemp_C) -> [VHAL_NVMLFWheelTemp_C]
  NVM1/15(VHAL_NVMRFWheelTemp_C) -> [VHAL_NVMRFWheelTemp_C]
  NVM1/16(VHAL_NVMLRWheelTemp_C) -> [VHAL_NVMLRWheelTemp_C]
  NVM1/17(VHAL_NVMRRWheelTemp_C) -> [VHAL_NVMRRWheelTemp_C]
  NVM1/18(VHAL_NVMFlashS1ID_raw) -> [VHAL_NVMFlashS1ID_raw]
  NVM1/19(VHAL_NVMFlashS2ID_raw) -> [VHAL_NVMFlashS2ID_raw]
  NVM1/20(VHAL_NVMFlashS3ID_raw) -> [VHAL_NVMFlashS3ID_raw]
  VOUTP_EAPS1MIN_pct/1 -> Data Type Conversion2/1
  VOUTP_EAPS2MIN_pct/1 -> Data Type Conversion3/1
  Multiply/1 -> Data Type Conversion127/1
  Data Type Conversion126/1 -> Mux/115
  Data Type Conversion129/1 -> Mux/113
  Data Type Conversion125/1 -> Mux/114
  Shift Arithmetic37/1 -> Data Type Conversion125/1
  Shift Arithmetic38/1 -> Data Type Conversion126/1
  Data Type Conversion128/1 -> Mux/112
  Bitwise AND48/1 -> Data Type Conversion128/1
  Bitwise AND49/1 -> Shift Arithmetic36/1
  Data Type Conversion127/1 -> Bitwise AND51/1, Bitwise AND50/1, Bitwise AND49/1, Bitwise AND48/1
  Shift Arithmetic36/1 -> Data Type Conversion129/1
  Bitwise AND51/1 -> Shift Arithmetic38/1
  Bitwise AND50/1 -> Shift Arithmetic37/1
  Data Type Conversion2/1 -> Multiply/1
  Bitwise AND54/1 -> Shift Arithmetic40/1
  Bitwise AND55/1 -> Shift Arithmetic41/1
  Shift Arithmetic39/1 -> Data Type Conversion133/1
  Data Type Conversion131/1 -> Bitwise AND52/1, Bitwise AND53/1, Bitwise AND54/1, Bitwise AND55/1
  Bitwise AND53/1 -> Shift Arithmetic39/1
  Bitwise AND52/1 -> Data Type Conversion132/1
  Shift Arithmetic41/1 -> Data Type Conversion130/1
  Shift Arithmetic40/1 -> Data Type Conversion44/1
  Multiply1/1 -> Data Type Conversion131/1
  Data Type Conversion132/1 -> Mux/116
  Data Type Conversion133/1 -> Mux/117
  Data Type Conversion44/1 -> Mux/118
  Data Type Conversion130/1 -> Mux/119
  Data Type Conversion3/1 -> Multiply1/1
  VOUTP_HoodSW_flg/1 -> Data Type Conversion134/1
  VOUTP_TailgateHDSW_flg/1 -> Data Type Conversion137/1
  VOUTP_CTDLockSW_flg/1 -> Data Type Conversion136/1
  VOUTP_TailgateSW_flg/1 -> Data Type Conversion135/1
  VOUTP_APMDoorControlSta_flg/1 -> Data Type Conversion138/1
  Data Type Conversion138/1 -> Mux/124
  VHAL_funAuto_flg/1 -> Data Type Conversion139/1
  VHAL_DiagDRLOFF_flg/1 -> Data Type Conversion140/1
  Data Type Conversion139/1 -> Mux/125
  Data Type Conversion140/1 -> Mux/126
  Data Type Conversion141/1 -> Mux/127
  Data Type Conversion142/1 -> Mux/128
  Data Type Conversion143/1 -> Mux/129
  Data Type Conversion144/1 -> Mux/130
  Data Type Conversion145/1 -> Mux/131
  Demux/1 -> Data Type Conversion146/1
  Demux/2 -> Data Type Conversion147/1
  Demux/3 -> Data Type Conversion148/1
  Demux/4 -> Data Type Conversion149/1
  Demux/5 -> Data Type Conversion150/1
  Demux/6 -> Data Type Conversion151/1
  Demux/7 -> Data Type Conversion152/1
  Demux/8 -> Data Type Conversion153/1
  VHAL_USSConfig_raw8/1 -> Demux/1
  Data Type Conversion146/1 -> Mux/132
  Data Type Conversion147/1 -> Mux/133
  Data Type Conversion148/1 -> Mux/134
  Data Type Conversion149/1 -> Mux/135
  Data Type Conversion150/1 -> Mux/136
  Data Type Conversion151/1 -> Mux/137
  Data Type Conversion152/1 -> Mux/138
  Data Type Conversion153/1 -> Mux/139
  Demux/16 -> Data Type Conversion161/1
  Demux/15 -> Data Type Conversion160/1
  Demux/14 -> Data Type Conversion159/1
  Demux/13 -> Data Type Conversion158/1
  Demux/12 -> Data Type Conversion157/1
  Demux/11 -> Data Type Conversion156/1
  Demux/10 -> Data Type Conversion155/1
  Demux/9 -> Data Type Conversion154/1
  Data Type Conversion154/1 -> Mux/140
  Data Type Conversion155/1 -> Mux/141
  Data Type Conversion156/1 -> Mux/142
  Data Type Conversion157/1 -> Mux/143
  Data Type Conversion158/1 -> Mux/144
  Data Type Conversion159/1 -> Mux/145
  Data Type Conversion160/1 -> Mux/146
  Data Type Conversion161/1 -> Mux/147
  Data Type Conversion177/1 -> Mux/163
  Data Type Conversion176/1 -> Mux/162
  Data Type Conversion175/1 -> Mux/161
  Data Type Conversion174/1 -> Mux/160
  Data Type Conversion173/1 -> Mux/159
  Data Type Conversion172/1 -> Mux/158
  Data Type Conversion171/1 -> Mux/157
  Data Type Conversion170/1 -> Mux/156
  Demux1/9 -> Data Type Conversion170/1
  Demux1/10 -> Data Type Conversion171/1
  Demux1/11 -> Data Type Conversion172/1
  Demux1/12 -> Data Type Conversion173/1
  Demux1/13 -> Data Type Conversion174/1
  Demux1/14 -> Data Type Conversion175/1
  Demux1/15 -> Data Type Conversion176/1
  Demux1/16 -> Data Type Conversion177/1
  Data Type Conversion169/1 -> Mux/155
  Data Type Conversion168/1 -> Mux/154
  Data Type Conversion167/1 -> Mux/153
  Data Type Conversion166/1 -> Mux/152
  Data Type Conversion165/1 -> Mux/151
  Data Type Conversion164/1 -> Mux/150
  Data Type Conversion163/1 -> Mux/149
  Data Type Conversion162/1 -> Mux/148
  VHAL_TireSize_raw8/1 -> Demux1/1
  Demux1/8 -> Data Type Conversion169/1
  Demux1/7 -> Data Type Conversion168/1
  Demux1/6 -> Data Type Conversion167/1
  Demux1/5 -> Data Type Conversion166/1
  Demux1/4 -> Data Type Conversion165/1
  Demux1/3 -> Data Type Conversion164/1
  Demux1/2 -> Data Type Conversion163/1
  Demux1/1 -> Data Type Conversion162/1
  Demux2/1 -> Data Type Conversion178/1
  Demux2/2 -> Data Type Conversion179/1
  Demux2/3 -> Data Type Conversion180/1
  Demux2/4 -> Data Type Conversion181/1
  Demux2/5 -> Data Type Conversion182/1
  Demux2/6 -> Data Type Conversion183/1
  Demux2/7 -> Data Type Conversion184/1
  Demux2/8 -> Data Type Conversion185/1
  VHAL_APSFunConfig_raw8/1 -> Demux2/1
  Data Type Conversion178/1 -> Mux/164
  Data Type Conversion179/1 -> Mux/165
  Data Type Conversion180/1 -> Mux/166
  Data Type Conversion181/1 -> Mux/167
  Data Type Conversion182/1 -> Mux/168
  Data Type Conversion183/1 -> Mux/169
  Data Type Conversion184/1 -> Mux/170
  Data Type Conversion185/1 -> Mux/171
  Demux2/16 -> Data Type Conversion193/1
  Demux2/15 -> Data Type Conversion192/1
  Demux2/14 -> Data Type Conversion191/1
  Demux2/13 -> Data Type Conversion190/1
  Demux2/12 -> Data Type Conversion189/1
  Demux2/11 -> Data Type Conversion188/1
  Demux2/10 -> Data Type Conversion187/1
  Demux2/9 -> Data Type Conversion186/1
  Data Type Conversion186/1 -> Mux/172
  Data Type Conversion187/1 -> Mux/173
  Data Type Conversion188/1 -> Mux/174
  Data Type Conversion189/1 -> Mux/175
  Data Type Conversion190/1 -> Mux/176
  Data Type Conversion191/1 -> Mux/177
  Data Type Conversion192/1 -> Mux/178
  Data Type Conversion193/1 -> Mux/179
  VOUTP_fUnlockSingle_flg/1 -> Data Type Conversion194/1
  Data Type Conversion194/1 -> Mux/180
  Gain3/1 -> Data Type Conversion145/1
  Gain2/1 -> Data Type Conversion144/1
  Gain1/1 -> Data Type Conversion143/1
  Gain/1 -> Data Type Conversion142/1
  Subsystem/1(Out1) -> Data Type Conversion141/1
  VHAL_DiagFMHT_s/1 -> Subsystem/1(VOUTP_DiagFMHT_s)
  VHAL_DiagFRTC_mA/1 -> Gain1/1
  VHAL_DiagRLTC_mA/1 -> Gain2/1
  VHAL_DiagRRTC_mA/1 -> Gain3/1
  VHAL_DiagFLTC_mA/1 -> Gain/1
  VOUTP_SaveRegenMode_enum/1 -> Data Type Conversion195/1
  Data Type Conversion195/1 -> Mux/181
  Data Type Conversion212/1 -> Mux/198
  VOUTP_AmbPwrWarnENFlash_enum/1 -> Data Type Conversion200/1
  Data Type Conversion197/1 -> Mux/183
  Data Type Conversion199/1 -> Mux/185
  VOUTP_AmbColorSta5_enum/1 -> Data Type Conversion206/1
  VOUTP_AmbBrightnessSta1_enum/1 -> Data Type Conversion208/1
  VOUTP_AmbBrightnessSta3_enum/1 -> Data Type Conversion210/1
  Data Type Conversion213/1 -> Mux/199
  Data Type Conversion196/1 -> Mux/182
  Data Type Conversion202/1 -> Mux/188
  Data Type Conversion200/1 -> Mux/186
  VOUTP_AmbBrightnessSta2_enum/1 -> Data Type Conversion209/1
  Data Type Conversion209/1 -> Mux/195
  Data Type Conversion201/1 -> Mux/187
  VOUTP_AmbColorSta3_enum/1 -> Data Type Conversion204/1
  VOUTP_AmbColorSta1_enum/1 -> Data Type Conversion202/1
  VOUTP_AmbBrightnessSta7_enum/1 -> Data Type Conversion213/1
  VOUTP_AmbColorSta4_enum/1 -> Data Type Conversion205/1
  VOUTP_AmbODAENFlash_enum/1 -> Data Type Conversion201/1
  VOUTP_AmbLinkDriStaFlash_enum/1 -> Data Type Conversion199/1
  VOUTP_AmbFunENFlash_enum/1 -> Data Type Conversion196/1
  Data Type Conversion204/1 -> Mux/190
  Data Type Conversion203/1 -> Mux/189
  VOUTP_AmbDimENFlash_enum/1 -> Data Type Conversion198/1
  VOUTP_AmbColorSta2_enum/1 -> Data Type Conversion203/1
  VOUTP_AmbColorSta7_enum/1 -> Data Type Conversion207/1
  Data Type Conversion208/1 -> Mux/194
  VOUTP_AmbWelENFlash_enum/1 -> Data Type Conversion197/1
  Data Type Conversion205/1 -> Mux/191
  VOUTP_AmbBrightnessSta4_enum/1 -> Data Type Conversion211/1
  Data Type Conversion207/1 -> Mux/193
  Data Type Conversion211/1 -> Mux/197
  Data Type Conversion210/1 -> Mux/196
  Data Type Conversion206/1 -> Mux/192
  VOUTP_AmbBrightnessSta5_enum/1 -> Data Type Conversion212/1
  Data Type Conversion198/1 -> Mux/184
  VOUTP_FDCTHCLEVentYSta_enum/1 -> Data Type Conversion224/1
  Data Type Conversion232/1 -> Mux/218
  VOUTP_LVentEN_flg/1 -> Data Type Conversion223/1
  Data Type Conversion233/1 -> Mux/219
  VOUTP_FDCTHCCLEVentYSta_enum/1 -> Data Type Conversion226/1
  Data Type Conversion231/1 -> Mux/217
  Data Type Conversion224/1 -> Mux/210
  VOUTP_FDCTHCLEVentZSta_enum/1 -> Data Type Conversion219/1
  VOUTP_CRVentEN_flg/1 -> Data Type Conversion229/1
  VOUTP_FDCFGSIONSWSta_flg/1 -> Data Type Conversion233/1
  Data Type Conversion227/1 -> Mux/213
  VOUTP_FDCFGSAirIntSta_enum/1 -> Data Type Conversion231/1
  VOUTP_FDCFGSChSta_enum/1 -> Data Type Conversion232/1
  VOUTP_RVentEN_flg/1 -> Data Type Conversion227/1
  VOUTP_FDCTHCCREVentYSta_enum/1 -> Data Type Conversion230/1
  VOUTP_FDCTHCCREVentZSta_enum/1 -> Data Type Conversion222/1
  VOUTP_FDCTHCCLEVentZSta_enum/1 -> Data Type Conversion220/1
  Data Type Conversion217/1 -> Mux/203
  VOUTP_FDCTHCREVentModeSta_enum/1 -> Data Type Conversion217/1
  Data Type Conversion214/1 -> Mux/200
  VOUTP_TurnSwTimeSetSta457_enum/1 -> Data Type Conversion215/1
  VOUTP_FDCTHCLEVentModeSta_enum/1 -> Data Type Conversion218/1
  Data Type Conversion230/1 -> Mux/216
  VOUTP_CLVentEN_flg/1 -> Data Type Conversion225/1
  Data Type Conversion215/1 -> Mux/201
  VOUTP_FDCTHCREVentZSta_enum/1 -> Data Type Conversion221/1
  VOUTP_FDCTHCREVentYSta_enum/1 -> Data Type Conversion228/1
  VOUTP_TurnSwTimeSetSta123_enum/1 -> Data Type Conversion214/1
  Data Type Conversion221/1 -> Mux/207
  Data Type Conversion218/1 -> Mux/204
  Data Type Conversion219/1 -> Mux/205
  Data Type Conversion223/1 -> Mux/209
  Data Type Conversion226/1 -> Mux/212
  Data Type Conversion229/1 -> Mux/215
  Data Type Conversion222/1 -> Mux/208
  Data Type Conversion220/1 -> Mux/206
  VOUTP_FDCTHCAirIntZ3Sta_enum/1 -> Data Type Conversion216/1
  Data Type Conversion225/1 -> Mux/211
  Data Type Conversion228/1 -> Mux/214
  Data Type Conversion216/1 -> Mux/202
  VOUTP_WalkOutLkENFunSta_flg/1 -> Data Type Conversion234/1
  VOUTP_WalkInUnLkENFunSta_flg/1 -> Data Type Conversion235/1
  VOUTP_FollowMeENFunSta_flg/1 -> Data Type Conversion237/1
  Data Type Conversion234/1 -> Mux/220
  Data Type Conversion235/1 -> Mux/221
  Data Type Conversion237/1 -> Mux/222
  Data Type Conversion236/1 -> Bitwise AND57/1, Bitwise AND56/1
  Shift Arithmetic42/1 -> Data Type Conversion239/1
  Bitwise AND56/1 -> Data Type Conversion238/1
  Bitwise AND57/1 -> Shift Arithmetic42/1
  Data Type Conversion238/1 -> Mux/223
  Data Type Conversion239/1 -> Mux/224
  Bitwise AND59/1 -> Shift Arithmetic43/1
  Bitwise AND58/1 -> Data Type Conversion241/1
  Shift Arithmetic43/1 -> Data Type Conversion242/1
  Data Type Conversion240/1 -> Bitwise AND58/1, Bitwise AND59/1
  Data Type Conversion243/1 -> Bitwise AND61/1, Bitwise AND60/1
  Shift Arithmetic44/1 -> Data Type Conversion245/1
  Bitwise AND60/1 -> Data Type Conversion244/1
  Bitwise AND61/1 -> Shift Arithmetic44/1
  Bitwise AND67/1 -> Shift Arithmetic47/1
  Bitwise AND66/1 -> Data Type Conversion253/1
  Shift Arithmetic47/1 -> Data Type Conversion254/1
  Data Type Conversion252/1 -> Bitwise AND66/1, Bitwise AND67/1
  Data Type Conversion249/1 -> Bitwise AND65/1, Bitwise AND64/1
  Shift Arithmetic46/1 -> Data Type Conversion251/1
  Bitwise AND64/1 -> Data Type Conversion250/1
  Bitwise AND65/1 -> Shift Arithmetic46/1
  Bitwise AND63/1 -> Shift Arithmetic45/1
  Bitwise AND62/1 -> Data Type Conversion247/1
  Shift Arithmetic45/1 -> Data Type Conversion248/1
  Data Type Conversion246/1 -> Bitwise AND62/1, Bitwise AND63/1
  Data Type Conversion241/1 -> Mux/225
  Data Type Conversion242/1 -> Mux/226
  Data Type Conversion244/1 -> Mux/227
  Data Type Conversion245/1 -> Mux/228
  Data Type Conversion247/1 -> Mux/229
  Data Type Conversion248/1 -> Mux/230
  Data Type Conversion250/1 -> Mux/231
  Data Type Conversion251/1 -> Mux/232
  Data Type Conversion253/1 -> Mux/233
  Data Type Conversion254/1 -> Mux/234
  VOUTP_PTGUserHeight1_cnt/1 -> Data Type Conversion236/1
  VOUTP_PTGUserHeight2_cnt/1 -> Data Type Conversion240/1
  VOUTP_PTGUserHeight3_cnt/1 -> Data Type Conversion243/1
  VOUTP_PTGUserHeight4_cnt/1 -> Data Type Conversion246/1
  VOUTP_PTGUserHeight5_cnt/1 -> Data Type Conversion249/1
  VOUTP_PTGUserHeight7_cnt/1 -> Data Type Conversion252/1
  VOUTP_PTGOpenHeight12_enum/1 -> Data Type Conversion255/1
  VOUTP_PTGOpenHeight34_enum/1 -> Data Type Conversion256/1
  VOUTP_PTGOpenHeight57_enum/1 -> Data Type Conversion257/1
  Data Type Conversion256/1 -> Mux/236
  Data Type Conversion257/1 -> Mux/237
  Bus Selector2/2 -> Data Type Conversion259/1  "<VHAL_WipRLSCmdHoldFilter_raw>"
  Bus Selector2/3 -> Data Type Conversion260/1  "<VHAL_WipRLSCmdCutFilter_raw>"
  Bus Selector2/1 -> Data Type Conversion258/1  "<VHAL_AutoWipHSpdEN_raw>"
  BHAL_DIDGetData_raw/1 -> Bus Selector2/1
  Data Type Conversion265/1 -> Mux/240
  VOUTP_ACCLevelMem57_enum/1 -> Data Type Conversion265/1
  Data Type Conversion264/1 -> Mux/239
  Data Type Conversion263/1 -> Mux/238
  VOUTP_ACCLevelMem12_enum/1 -> Data Type Conversion263/1
  VOUTP_ACCLevelMem34_enum/1 -> Data Type Conversion264/1
  Data Type Conversion258/1 -> Mux/241
  Data Type Conversion259/1 -> Mux/242
  Data Type Conversion260/1 -> Mux/243
  VOUTP_AutoLockMem_enum/1 -> Data Type Conversion261/1
  Data Type Conversion261/1 -> Mux/244
  VOUTP_AutoUnlockMem_enum/1 -> Data Type Conversion262/1
  Data Type Conversion262/1 -> Mux/245
  Mux/1 -> [HAL_NvmWriteData256BytesArray1_raw]
  Mux1/1 -> [HAL_NvmWriteData256BytesArray2_raw]
  [HAL_NvmWriteData256BytesArray1_raw] -> Mux2/1
  Mux2/1 -> HAL_NvmWriteData_raw/1
  [HAL_NvmWriteData256BytesArray3_raw] -> Mux2/3
  [HAL_NvmWriteData256BytesArray4_raw] -> Mux2/4
  Mux3/1 -> [HAL_NvmWriteData256BytesArray3_raw]
  Constant/1 -> [HAL_NvmWriteData256BytesArray4_raw]
  [HAL_NvmWriteData256BytesArray2_raw] -> Mux2/2
  Bitwise AND69/1 -> Shift Arithmetic48/1
  Data Type Conversion267/1 -> Mux/246
  VOUTP_MILDIST_km/1 -> Data Type Conversion266/1
  Data Type Conversion268/1 -> Mux/247
  Data Type Conversion266/1 -> Bitwise AND68/1, Bitwise AND69/1
  Shift Arithmetic48/1 -> Data Type Conversion268/1
  Bitwise AND68/1 -> Data Type Conversion267/1
  VOUTP_WARMUPS_cnt/1 -> Data Type Conversion269/1
  Data Type Conversion269/1 -> Mux/248
  Bitwise AND70/1 -> Data Type Conversion271/1
  Shift Arithmetic49/1 -> Data Type Conversion272/1
  Data Type Conversion270/1 -> Bitwise AND71/1, Bitwise AND70/1
  VOUTP_CLRDIST_km/1 -> Data Type Conversion270/1
  Bitwise AND71/1 -> Shift Arithmetic49/1
  Data Type Conversion271/1 -> Mux/249
  Data Type Conversion272/1 -> Mux/250
  Data Type Conversion275/1 -> Mux/252
  Data Type Conversion274/1 -> Mux/251
  Bitwise AND73/1 -> Shift Arithmetic50/1
  VOUTP_MILTIME_min/1 -> Data Type Conversion273/1
  Data Type Conversion273/1 -> Bitwise AND72/1, Bitwise AND73/1
  Shift Arithmetic50/1 -> Data Type Conversion275/1
  Bitwise AND72/1 -> Data Type Conversion274/1
  Bitwise AND74/1 -> Data Type Conversion277/1
  Shift Arithmetic51/1 -> Data Type Conversion278/1
  Data Type Conversion276/1 -> Bitwise AND75/1, Bitwise AND74/1
  VOUTP_CLRTIME_min/1 -> Data Type Conversion276/1
  Bitwise AND75/1 -> Shift Arithmetic51/1
  Data Type Conversion277/1 -> Mux/253
  Data Type Conversion278/1 -> Mux/254
  Data Type Conversion279/1 -> Bitwise AND76/1, Bitwise AND77/1, Bitwise AND78/1, Bitwise AND79/1
  Bitwise AND76/1 -> Data Type Conversion281/1
  Bitwise AND77/1 -> Shift Arithmetic52/1
  Shift Arithmetic54/1 -> Data Type Conversion280/1
  Bitwise AND78/1 -> Shift Arithmetic53/1
  Bitwise AND79/1 -> Shift Arithmetic54/1
  Shift Arithmetic52/1 -> Data Type Conversion282/1
  Shift Arithmetic53/1 -> Data Type Conversion283/1
  Data Type Conversion286/1 -> Mux/256
  Data Type Conversion285/1 -> Mux/255
  Bitwise AND81/1 -> Shift Arithmetic55/1
  VOUTP_NUMPSATRIPSFLTMEMCLR_cnt/1 -> Data Type Conversion284/1
  Data Type Conversion284/1 -> Bitwise AND80/1, Bitwise AND81/1
  Shift Arithmetic55/1 -> Data Type Conversion286/1
  Bitwise AND80/1 -> Data Type Conversion285/1
  Bitwise AND85/1 -> Shift Arithmetic58/1
  Shift Arithmetic56/1 -> Data Type Conversion290/1
  Shift Arithmetic57/1 -> Data Type Conversion291/1
  Bitwise AND84/1 -> Shift Arithmetic57/1
  Bitwise AND83/1 -> Shift Arithmetic56/1
  Bitwise AND82/1 -> Data Type Conversion289/1
  Shift Arithmetic58/1 -> Data Type Conversion288/1
  Data Type Conversion287/1 -> Bitwise AND82/1, Bitwise AND83/1, Bitwise AND84/1, Bitwise AND85/1
  VOUTP_PSAR_sec/1 -> Data Type Conversion287/1
  VOUTP_PSAL_sec/1 -> Data Type Conversion292/1
  Data Type Conversion292/1 -> Bitwise AND89/1, Bitwise AND88/1, Bitwise AND87/1, Bitwise AND86/1
  Shift Arithmetic61/1 -> Data Type Conversion293/1
  Bitwise AND86/1 -> Data Type Conversion294/1
  Bitwise AND87/1 -> Shift Arithmetic59/1
  Bitwise AND88/1 -> Shift Arithmetic60/1
  Shift Arithmetic60/1 -> Data Type Conversion296/1
  Shift Arithmetic59/1 -> Data Type Conversion295/1
  Bitwise AND89/1 -> Shift Arithmetic61/1
  Bitwise AND97/1 -> Shift Arithmetic67/1
  Shift Arithmetic65/1 -> Data Type Conversion305/1
  Shift Arithmetic66/1 -> Data Type Conversion306/1
  Bitwise AND96/1 -> Shift Arithmetic66/1
  Bitwise AND95/1 -> Shift Arithmetic65/1
  Bitwise AND94/1 -> Data Type Conversion304/1
  Shift Arithmetic67/1 -> Data Type Conversion303/1
  Data Type Conversion302/1 -> Bitwise AND94/1, Bitwise AND95/1, Bitwise AND96/1, Bitwise AND97/1
  VOUTP_IPSAL_sec/1 -> Data Type Conversion302/1
  VOUTP_IPSAR_sec/1 -> Data Type Conversion297/1
  Data Type Conversion297/1 -> Bitwise AND93/1, Bitwise AND92/1, Bitwise AND91/1, Bitwise AND90/1
  Shift Arithmetic64/1 -> Data Type Conversion298/1
  Bitwise AND90/1 -> Data Type Conversion299/1
  Bitwise AND91/1 -> Shift Arithmetic62/1
  Bitwise AND92/1 -> Shift Arithmetic63/1
  Shift Arithmetic63/1 -> Data Type Conversion301/1
  Shift Arithmetic62/1 -> Data Type Conversion300/1
  Bitwise AND93/1 -> Shift Arithmetic64/1
  Bitwise AND101/1 -> Shift Arithmetic70/1
  Shift Arithmetic68/1 -> Data Type Conversion310/1
  Shift Arithmetic69/1 -> Data Type Conversion311/1
  Bitwise AND100/1 -> Shift Arithmetic69/1
  Bitwise AND99/1 -> Shift Arithmetic68/1
  Bitwise AND98/1 -> Data Type Conversion309/1
  Shift Arithmetic70/1 -> Data Type Conversion308/1
  Data Type Conversion307/1 -> Bitwise AND98/1, Bitwise AND99/1, Bitwise AND100/1, Bitwise AND101/1
  VOUTP_CPSAR_sec/1 -> Data Type Conversion307/1
  VOUTP_CPSAL_sec/1 -> Data Type Conversion312/1
  Data Type Conversion312/1 -> Bitwise AND105/1, Bitwise AND104/1, Bitwise AND103/1, Bitwise AND102/1
  Shift Arithmetic73/1 -> Data Type Conversion313/1
  Bitwise AND102/1 -> Data Type Conversion314/1
  Bitwise AND103/1 -> Shift Arithmetic71/1
  Bitwise AND104/1 -> Shift Arithmetic72/1
  Shift Arithmetic72/1 -> Data Type Conversion316/1
  Shift Arithmetic71/1 -> Data Type Conversion315/1
  Bitwise AND105/1 -> Shift Arithmetic73/1
  Data Type Conversion281/1 -> Mux1/1
  Data Type Conversion282/1 -> Mux1/2
  Data Type Conversion283/1 -> Mux1/3
  Data Type Conversion280/1 -> Mux1/4
  Data Type Conversion289/1 -> Mux1/5
  Data Type Conversion290/1 -> Mux1/6
  Data Type Conversion291/1 -> Mux1/7
  Data Type Conversion288/1 -> Mux1/8
  Data Type Conversion294/1 -> Mux1/9
  Data Type Conversion295/1 -> Mux1/10
  Data Type Conversion296/1 -> Mux1/11
  Data Type Conversion293/1 -> Mux1/12
  Data Type Conversion299/1 -> Mux1/13
  Data Type Conversion300/1 -> Mux1/14
  Data Type Conversion301/1 -> Mux1/15
  Data Type Conversion298/1 -> Mux1/16
  Data Type Conversion304/1 -> Mux1/17
  Data Type Conversion305/1 -> Mux1/18
  Data Type Conversion306/1 -> Mux1/19
  Data Type Conversion303/1 -> Mux1/20
  Data Type Conversion309/1 -> Mux1/21
  Data Type Conversion310/1 -> Mux1/22
  Data Type Conversion311/1 -> Mux1/23
  Data Type Conversion308/1 -> Mux1/24
  Data Type Conversion314/1 -> Mux1/25
  Data Type Conversion315/1 -> Mux1/26
  Data Type Conversion316/1 -> Mux1/27
  Data Type Conversion313/1 -> Mux1/28
  convert_in1/1 -> Data Type Conversion317/1
  Data Type Conversion318/1 -> Mux1/32
  Data Type Conversion321/1 -> Mux1/31
  Data Type Conversion320/1 -> Mux1/30
  Data Type Conversion319/1 -> Mux1/29
  Bitwise AND109/1 -> Shift Arithmetic76/1
  Shift Arithmetic74/1 -> Data Type Conversion320/1
  Shift Arithmetic75/1 -> Data Type Conversion321/1
  Bitwise AND108/1 -> Shift Arithmetic75/1
  Bitwise AND107/1 -> Shift Arithmetic74/1
  Bitwise AND106/1 -> Data Type Conversion319/1
  Shift Arithmetic76/1 -> Data Type Conversion318/1
  Data Type Conversion317/1 -> Bitwise AND107/1, Bitwise AND108/1, Bitwise AND109/1, Bitwise AND106/1
  Data Type Conversion322/1 -> Bitwise AND110/1, Bitwise AND113/1, Bitwise AND112/1, Bitwise AND111/1
  Shift Arithmetic79/1 -> Data Type Conversion323/1
  Bitwise AND110/1 -> Data Type Conversion324/1
  Bitwise AND111/1 -> Shift Arithmetic77/1
  Bitwise AND112/1 -> Shift Arithmetic78/1
  Shift Arithmetic78/1 -> Data Type Conversion326/1
  Shift Arithmetic77/1 -> Data Type Conversion325/1
  Bitwise AND113/1 -> Shift Arithmetic79/1
  Data Type Conversion325/1 -> Mux1/34
  Data Type Conversion326/1 -> Mux1/35
  Data Type Conversion323/1 -> Mux1/36
  convert_in2/1 -> Data Type Conversion322/1
  VOUTP_HVBNE_kWh/1 -> convert_in2/1
  Data Type Conversion324/1 -> Mux1/33
  Data Type Conversion328/1 -> Mux1/37
  Shift Arithmetic80/1 -> Data Type Conversion329/1
  Data Type Conversion329/1 -> Mux1/38
  Bitwise AND114/1 -> Data Type Conversion328/1
  VOUTP_IGNCNTR_cnt/1 -> Data Type Conversion327/1
  Data Type Conversion327/1 -> Bitwise AND114/1, Bitwise AND115/1
  Bitwise AND115/1 -> Shift Arithmetic80/1
  Data Type Conversion332/1 -> Mux1/39
  VOUTP_TNBCPSAR_Ahr/1 -> convert_in3/1
  Data Type Conversion331/1 -> Mux1/42
  Data Type Conversion334/1 -> Mux1/41
  Data Type Conversion333/1 -> Mux1/40
  Bitwise AND119/1 -> Shift Arithmetic83/1
  Shift Arithmetic81/1 -> Data Type Conversion333/1
  Shift Arithmetic82/1 -> Data Type Conversion334/1
  Bitwise AND118/1 -> Shift Arithmetic82/1
  Bitwise AND117/1 -> Shift Arithmetic81/1
  Bitwise AND116/1 -> Data Type Conversion332/1
  Shift Arithmetic83/1 -> Data Type Conversion331/1
  Data Type Conversion330/1 -> Bitwise AND117/1, Bitwise AND118/1, Bitwise AND119/1, Bitwise AND116/1
  Data Type Conversion335/1 -> Bitwise AND120/1, Bitwise AND123/1, Bitwise AND122/1, Bitwise AND121/1
  Shift Arithmetic86/1 -> Data Type Conversion336/1
  Bitwise AND120/1 -> Data Type Conversion337/1
  Bitwise AND121/1 -> Shift Arithmetic84/1
  Bitwise AND122/1 -> Shift Arithmetic85/1
  Shift Arithmetic85/1 -> Data Type Conversion339/1
  Shift Arithmetic84/1 -> Data Type Conversion338/1
  Bitwise AND123/1 -> Shift Arithmetic86/1
  Data Type Conversion338/1 -> Mux1/44
  Data Type Conversion339/1 -> Mux1/45
  Data Type Conversion336/1 -> Mux1/46
  convert_in4/1 -> Data Type Conversion335/1
  VOUTP_TNBCPSAL_Ahr/1 -> convert_in4/1
  Data Type Conversion337/1 -> Mux1/43
  Data Type Conversion342/1 -> Mux1/47
  VOUTP_TNECPSAR_kWh/1 -> convert_in5/1
  convert_in5/1 -> Data Type Conversion340/1
  Data Type Conversion341/1 -> Mux1/50
  Data Type Conversion344/1 -> Mux1/49
  Data Type Conversion343/1 -> Mux1/48
  Bitwise AND127/1 -> Shift Arithmetic89/1
  Shift Arithmetic87/1 -> Data Type Conversion343/1
  Shift Arithmetic88/1 -> Data Type Conversion344/1
  Bitwise AND126/1 -> Shift Arithmetic88/1
  Bitwise AND125/1 -> Shift Arithmetic87/1
  Bitwise AND124/1 -> Data Type Conversion342/1
  Shift Arithmetic89/1 -> Data Type Conversion341/1
  Data Type Conversion340/1 -> Bitwise AND125/1, Bitwise AND126/1, Bitwise AND127/1, Bitwise AND124/1
  Data Type Conversion345/1 -> Bitwise AND128/1, Bitwise AND131/1, Bitwise AND130/1, Bitwise AND129/1
  Shift Arithmetic92/1 -> Data Type Conversion346/1
  Bitwise AND128/1 -> Data Type Conversion347/1
  Bitwise AND129/1 -> Shift Arithmetic90/1
  Bitwise AND130/1 -> Shift Arithmetic91/1
  Shift Arithmetic91/1 -> Data Type Conversion349/1
  Shift Arithmetic90/1 -> Data Type Conversion348/1
  Bitwise AND131/1 -> Shift Arithmetic92/1
  Data Type Conversion348/1 -> Mux1/52
  Data Type Conversion349/1 -> Mux1/53
  Data Type Conversion346/1 -> Mux1/54
  convert_in6/1 -> Data Type Conversion345/1
  VOUTP_TNECPSAL_kWh/1 -> convert_in6/1
  Data Type Conversion347/1 -> Mux1/51
  Data Type Conversion352/1 -> Mux1/55
  VOUTP_TEBPSAR_kWh/1 -> convert_in7/1
  convert_in7/1 -> Data Type Conversion350/1
  Data Type Conversion351/1 -> Mux1/58
  Data Type Conversion354/1 -> Mux1/57
  Data Type Conversion353/1 -> Mux1/56
  Bitwise AND135/1 -> Shift Arithmetic95/1
  Shift Arithmetic93/1 -> Data Type Conversion353/1
  Shift Arithmetic94/1 -> Data Type Conversion354/1
  Bitwise AND134/1 -> Shift Arithmetic94/1
  Bitwise AND133/1 -> Shift Arithmetic93/1
  Bitwise AND132/1 -> Data Type Conversion352/1
  Shift Arithmetic95/1 -> Data Type Conversion351/1
  Data Type Conversion350/1 -> Bitwise AND133/1, Bitwise AND134/1, Bitwise AND135/1, Bitwise AND132/1
  Data Type Conversion355/1 -> Bitwise AND136/1, Bitwise AND139/1, Bitwise AND138/1, Bitwise AND137/1
  Shift Arithmetic98/1 -> Data Type Conversion356/1
  Bitwise AND136/1 -> Data Type Conversion357/1
  Bitwise AND137/1 -> Shift Arithmetic96/1
  Bitwise AND138/1 -> Shift Arithmetic97/1
  Shift Arithmetic97/1 -> Data Type Conversion359/1
  Shift Arithmetic96/1 -> Data Type Conversion358/1
  Bitwise AND139/1 -> Shift Arithmetic98/1
  Data Type Conversion358/1 -> Mux1/60
  Data Type Conversion359/1 -> Mux1/61
  Data Type Conversion356/1 -> Mux1/62
  convert_in8/1 -> Data Type Conversion355/1
  VOUTP_TEBPSAL_kWh/1 -> convert_in8/1
  Data Type Conversion357/1 -> Mux1/59
  Data Type Conversion362/1 -> Mux1/63
  VOUTP_TGEOVCR_kWh/1 -> convert_in9/1
  convert_in9/1 -> Data Type Conversion360/1
  Data Type Conversion361/1 -> Mux1/66
  Data Type Conversion364/1 -> Mux1/65
  Data Type Conversion363/1 -> Mux1/64
  Bitwise AND143/1 -> Shift Arithmetic101/1
  Shift Arithmetic99/1 -> Data Type Conversion363/1
  Shift Arithmetic100/1 -> Data Type Conversion364/1
  Bitwise AND142/1 -> Shift Arithmetic100/1
  Bitwise AND141/1 -> Shift Arithmetic99/1
  Bitwise AND140/1 -> Data Type Conversion362/1
  Shift Arithmetic101/1 -> Data Type Conversion361/1
  Data Type Conversion360/1 -> Bitwise AND141/1, Bitwise AND142/1, Bitwise AND143/1, Bitwise AND140/1
  Data Type Conversion365/1 -> Bitwise AND144/1, Bitwise AND147/1, Bitwise AND146/1, Bitwise AND145/1
  Shift Arithmetic103/1 -> Data Type Conversion366/1
  Bitwise AND144/1 -> Data Type Conversion367/1
  Bitwise AND145/1 -> Shift Arithmetic104/1
  Bitwise AND146/1 -> Shift Arithmetic102/1
  Shift Arithmetic102/1 -> Data Type Conversion369/1
  Shift Arithmetic104/1 -> Data Type Conversion368/1
  Bitwise AND147/1 -> Shift Arithmetic103/1
  Data Type Conversion368/1 -> Mux1/68
  Data Type Conversion369/1 -> Mux1/69
  Data Type Conversion366/1 -> Mux1/70
  convert_in10/1 -> Data Type Conversion365/1
  VOUTP_TGEOVCL_kWh/1 -> convert_in10/1
  Data Type Conversion367/1 -> Mux1/67
  Data Type Conversion372/1 -> Mux1/71
  VOUTP_GECHGOVCDCR_kWh/1 -> convert_in11/1
  convert_in11/1 -> Data Type Conversion370/1
  Data Type Conversion371/1 -> Mux1/74
  Data Type Conversion374/1 -> Mux1/73
  Data Type Conversion373/1 -> Mux1/72
  Bitwise AND151/1 -> Shift Arithmetic106/1
  Shift Arithmetic107/1 -> Data Type Conversion373/1
  Shift Arithmetic105/1 -> Data Type Conversion374/1
  Bitwise AND150/1 -> Shift Arithmetic105/1
  Bitwise AND149/1 -> Shift Arithmetic107/1
  Bitwise AND148/1 -> Data Type Conversion372/1
  Shift Arithmetic106/1 -> Data Type Conversion371/1
  Data Type Conversion370/1 -> Bitwise AND149/1, Bitwise AND150/1, Bitwise AND151/1, Bitwise AND148/1
  Data Type Conversion375/1 -> Bitwise AND152/1, Bitwise AND155/1, Bitwise AND154/1, Bitwise AND153/1
  Shift Arithmetic109/1 -> Data Type Conversion376/1
  Bitwise AND152/1 -> Data Type Conversion377/1
  Bitwise AND153/1 -> Shift Arithmetic110/1
  Bitwise AND154/1 -> Shift Arithmetic108/1
  Shift Arithmetic108/1 -> Data Type Conversion379/1
  Shift Arithmetic110/1 -> Data Type Conversion378/1
  Bitwise AND155/1 -> Shift Arithmetic109/1
  Data Type Conversion378/1 -> Mux1/76
  Data Type Conversion379/1 -> Mux1/77
  Data Type Conversion376/1 -> Mux1/78
  convert_in12/1 -> Data Type Conversion375/1
  Data Type Conversion377/1 -> Mux1/75
  VOUTP_GECHGOVCDCL_kWh/1 -> convert_in12/1
  Data Type Conversion382/1 -> Mux1/79
  convert_in16/1 -> Data Type Conversion380/1
  Data Type Conversion381/1 -> Mux1/82
  Data Type Conversion384/1 -> Mux1/81
  Data Type Conversion383/1 -> Mux1/80
  Bitwise AND159/1 -> Shift Arithmetic112/1
  Shift Arithmetic113/1 -> Data Type Conversion383/1
  Shift Arithmetic111/1 -> Data Type Conversion384/1
  Bitwise AND158/1 -> Shift Arithmetic111/1
  Bitwise AND157/1 -> Shift Arithmetic113/1
  Bitwise AND156/1 -> Data Type Conversion382/1
  Shift Arithmetic112/1 -> Data Type Conversion381/1
  Data Type Conversion380/1 -> Bitwise AND157/1, Bitwise AND158/1, Bitwise AND159/1, Bitwise AND156/1
  VOUTP_GECHGOVCACR_kWh/1 -> convert_in16/1
  Data Type Conversion385/1 -> Bitwise AND160/1, Bitwise AND163/1, Bitwise AND162/1, Bitwise AND161/1
  Shift Arithmetic115/1 -> Data Type Conversion386/1
  Bitwise AND160/1 -> Data Type Conversion387/1
  Bitwise AND161/1 -> Shift Arithmetic116/1
  Bitwise AND162/1 -> Shift Arithmetic114/1
  Shift Arithmetic114/1 -> Data Type Conversion389/1
  Shift Arithmetic116/1 -> Data Type Conversion388/1
  Bitwise AND163/1 -> Shift Arithmetic115/1
  Data Type Conversion388/1 -> Mux1/84
  Data Type Conversion389/1 -> Mux1/85
  Data Type Conversion386/1 -> Mux1/86
  convert_in13/1 -> Data Type Conversion385/1
  Data Type Conversion387/1 -> Mux1/83
  VOUTP_GECHGOVCACL_kWh/1 -> convert_in13/1
  VOUTP_RESSV2XENNONPSAR_kWh/1 -> convert_in14/1
  Data Type Conversion392/1 -> Mux1/87
  convert_in14/1 -> Data Type Conversion390/1
  Data Type Conversion391/1 -> Mux1/90
  Data Type Conversion394/1 -> Mux1/89
  Data Type Conversion393/1 -> Mux1/88
  Bitwise AND167/1 -> Shift Arithmetic118/1
  Shift Arithmetic119/1 -> Data Type Conversion393/1
  Shift Arithmetic117/1 -> Data Type Conversion394/1
  Bitwise AND166/1 -> Shift Arithmetic117/1
  Bitwise AND165/1 -> Shift Arithmetic119/1
  Bitwise AND164/1 -> Data Type Conversion392/1
  Shift Arithmetic118/1 -> Data Type Conversion391/1
  Data Type Conversion390/1 -> Bitwise AND165/1, Bitwise AND166/1, Bitwise AND167/1, Bitwise AND164/1
  Data Type Conversion395/1 -> Bitwise AND168/1, Bitwise AND171/1, Bitwise AND170/1, Bitwise AND169/1
  Shift Arithmetic121/1 -> Data Type Conversion396/1
  Bitwise AND168/1 -> Data Type Conversion397/1
  Bitwise AND169/1 -> Shift Arithmetic122/1
  Bitwise AND170/1 -> Shift Arithmetic120/1
  Shift Arithmetic120/1 -> Data Type Conversion399/1
  Shift Arithmetic122/1 -> Data Type Conversion398/1
  Bitwise AND171/1 -> Shift Arithmetic121/1
  Data Type Conversion398/1 -> Mux1/92
  Data Type Conversion399/1 -> Mux1/93
  Data Type Conversion396/1 -> Mux1/94
  convert_in15/1 -> Data Type Conversion395/1
  Data Type Conversion397/1 -> Mux1/91
  VOUTP_RESSV2XENNONPSAL_kWh/1 -> convert_in15/1
  VOUTP_ODOMETER_km/1 -> convert_in/1
  convert_in/1 -> Data Type Conversion279/1
  VOUTP_HVBNAH_Ahr/1 -> convert_in1/1
  convert_in3/1 -> Data Type Conversion330/1
  Data Type Conversion402/1 -> Mux1/95
  VOUTP_PKERNumerator_kphsqr/1 -> Data Type Conversion400/1
  Data Type Conversion401/1 -> Mux1/98
  Data Type Conversion404/1 -> Mux1/97
  Data Type Conversion403/1 -> Mux1/96
  Bitwise AND175/1 -> Shift Arithmetic124/1
  Shift Arithmetic125/1 -> Data Type Conversion403/1
  Shift Arithmetic123/1 -> Data Type Conversion404/1
  Bitwise AND174/1 -> Shift Arithmetic123/1
  Bitwise AND173/1 -> Shift Arithmetic125/1
  Bitwise AND172/1 -> Data Type Conversion402/1
  Shift Arithmetic124/1 -> Data Type Conversion401/1
  Data Type Conversion400/1 -> Bitwise AND173/1, Bitwise AND174/1, Bitwise AND175/1, Bitwise AND172/1
  Data Type Conversion405/1 -> Bitwise AND176/1, Bitwise AND179/1, Bitwise AND178/1, Bitwise AND177/1
  Shift Arithmetic127/1 -> Data Type Conversion406/1
  Bitwise AND176/1 -> Data Type Conversion407/1
  Bitwise AND177/1 -> Shift Arithmetic128/1
  Bitwise AND178/1 -> Shift Arithmetic126/1
  Shift Arithmetic126/1 -> Data Type Conversion409/1
  Shift Arithmetic128/1 -> Data Type Conversion408/1
  Bitwise AND179/1 -> Shift Arithmetic127/1
  Data Type Conversion408/1 -> Mux1/100
  Data Type Conversion409/1 -> Mux1/101
  Data Type Conversion406/1 -> Mux1/102
  VOUTP_PKELNumerator_kphsqr/1 -> Data Type Conversion405/1
  Data Type Conversion407/1 -> Mux1/99
  VOUTP_AvgBattTempPSAR_C/1 -> convert_in17/1
  convert_in17/1 -> Data Type Conversion410/1
  convert_in18/1 -> Data Type Conversion411/1
  VOUTP_AvgBattTempPSAL_C/1 -> convert_in18/1
  VOUTP_AvgBattTempOVCL_C/1 -> convert_in20/1
  convert_in20/1 -> Data Type Conversion413/1
  convert_in19/1 -> Data Type Conversion412/1
  VOUTP_AvgBattTempOVCR_C/1 -> convert_in19/1
  VOUTP_AvgBattTempOFFR_C/1 -> convert_in21/1
  convert_in21/1 -> Data Type Conversion414/1
  convert_in22/1 -> Data Type Conversion415/1
  VOUTP_AvgBattTempOFFL_C/1 -> convert_in22/1
  VOUTP_ResetCDEODTR_km/1 -> convert_in23/1
  Data Type Conversion418/1 -> Mux1/103
  Data Type Conversion417/1 -> Mux1/106
  Data Type Conversion420/1 -> Mux1/105
  Data Type Conversion419/1 -> Mux1/104
  Bitwise AND183/1 -> Shift Arithmetic130/1
  Shift Arithmetic131/1 -> Data Type Conversion419/1
  Shift Arithmetic129/1 -> Data Type Conversion420/1
  Bitwise AND182/1 -> Shift Arithmetic129/1
  Bitwise AND181/1 -> Shift Arithmetic131/1
  Bitwise AND180/1 -> Data Type Conversion418/1
  Shift Arithmetic130/1 -> Data Type Conversion417/1
  Data Type Conversion416/1 -> Bitwise AND181/1, Bitwise AND182/1, Bitwise AND183/1, Bitwise AND180/1
  convert_in23/1 -> Data Type Conversion416/1
  Data Type Conversion410/1 -> Mux1/107
  Data Type Conversion411/1 -> Mux1/108
  Data Type Conversion412/1 -> Mux1/109
  Data Type Conversion413/1 -> Mux1/110
  Data Type Conversion414/1 -> Mux1/111
  Data Type Conversion415/1 -> Mux1/112
  Data Type Conversion423/1 -> Mux1/113
  VOUTP_QTYPSATRIPSR_cnt/1 -> Data Type Conversion421/1
  Data Type Conversion422/1 -> Mux1/116
  Data Type Conversion425/1 -> Mux1/115
  Data Type Conversion424/1 -> Mux1/114
  Bitwise AND187/1 -> Shift Arithmetic133/1
  Shift Arithmetic134/1 -> Data Type Conversion424/1
  Shift Arithmetic132/1 -> Data Type Conversion425/1
  Bitwise AND186/1 -> Shift Arithmetic132/1
  Bitwise AND185/1 -> Shift Arithmetic134/1
  Bitwise AND184/1 -> Data Type Conversion423/1
  Shift Arithmetic133/1 -> Data Type Conversion422/1
  Data Type Conversion421/1 -> Bitwise AND185/1, Bitwise AND186/1, Bitwise AND187/1, Bitwise AND184/1
  Data Type Conversion426/1 -> Bitwise AND188/1, Bitwise AND191/1, Bitwise AND190/1, Bitwise AND189/1
  Shift Arithmetic136/1 -> Data Type Conversion427/1
  Bitwise AND188/1 -> Data Type Conversion428/1
  Bitwise AND189/1 -> Shift Arithmetic137/1
  Bitwise AND190/1 -> Shift Arithmetic135/1
  Shift Arithmetic135/1 -> Data Type Conversion430/1
  Shift Arithmetic137/1 -> Data Type Conversion429/1
  Bitwise AND191/1 -> Shift Arithmetic136/1
  Data Type Conversion429/1 -> Mux1/118
  Data Type Conversion430/1 -> Mux1/119
  Data Type Conversion427/1 -> Mux1/120
  VOUTP_QTYPSATRIPSL_cnt/1 -> Data Type Conversion426/1
  Data Type Conversion428/1 -> Mux1/117
  VOUTP_RESSCNTDODRNGR_cnt/1 -> Demux3/1
  Bitwise AND192/1 -> Data Type Conversion432/1
  Bitwise AND193/1 -> Shift Arithmetic138/1
  Data Type Conversion431/1 -> Bitwise AND192/1, Bitwise AND193/1
  Data Type Conversion433/1 -> Mux1/122
  Data Type Conversion432/1 -> Mux1/121
  Shift Arithmetic138/1 -> Data Type Conversion433/1
  Shift Arithmetic139/1 -> Data Type Conversion436/1
  Data Type Conversion435/1 -> Mux1/123
  Data Type Conversion436/1 -> Mux1/124
  Data Type Conversion434/1 -> Bitwise AND195/1, Bitwise AND194/1
  Bitwise AND195/1 -> Shift Arithmetic139/1
  Bitwise AND194/1 -> Data Type Conversion435/1
  Bitwise AND198/1 -> Data Type Conversion441/1
  Bitwise AND199/1 -> Shift Arithmetic141/1
  Data Type Conversion440/1 -> Bitwise AND198/1, Bitwise AND199/1
  Data Type Conversion442/1 -> Mux1/128
  Data Type Conversion441/1 -> Mux1/127
  Shift Arithmetic141/1 -> Data Type Conversion442/1
  Shift Arithmetic140/1 -> Data Type Conversion439/1
  Data Type Conversion438/1 -> Mux1/125
  Data Type Conversion439/1 -> Mux1/126
  Data Type Conversion437/1 -> Bitwise AND197/1, Bitwise AND196/1
  Bitwise AND197/1 -> Shift Arithmetic140/1
  Bitwise AND196/1 -> Data Type Conversion438/1
  Bitwise AND204/1 -> Data Type Conversion450/1
  Bitwise AND205/1 -> Shift Arithmetic144/1
  Data Type Conversion449/1 -> Bitwise AND204/1, Bitwise AND205/1
  Data Type Conversion451/1 -> Mux1/134
  Data Type Conversion450/1 -> Mux1/133
  Shift Arithmetic144/1 -> Data Type Conversion451/1
  Shift Arithmetic145/1 -> Data Type Conversion454/1
  Data Type Conversion453/1 -> Mux1/135
  Data Type Conversion454/1 -> Mux1/136
  Data Type Conversion452/1 -> Bitwise AND207/1, Bitwise AND206/1
  Bitwise AND207/1 -> Shift Arithmetic145/1
  Bitwise AND206/1 -> Data Type Conversion453/1
  Bitwise AND202/1 -> Data Type Conversion447/1
  Bitwise AND203/1 -> Shift Arithmetic143/1
  Data Type Conversion446/1 -> Bitwise AND202/1, Bitwise AND203/1
  Data Type Conversion448/1 -> Mux1/132
  Data Type Conversion447/1 -> Mux1/131
  Shift Arithmetic143/1 -> Data Type Conversion448/1
  Shift Arithmetic142/1 -> Data Type Conversion445/1
  Data Type Conversion444/1 -> Mux1/129
  Data Type Conversion445/1 -> Mux1/130
  Data Type Conversion443/1 -> Bitwise AND201/1, Bitwise AND200/1
  Bitwise AND201/1 -> Shift Arithmetic142/1
  Bitwise AND200/1 -> Data Type Conversion444/1
  Demux3/3 -> Data Type Conversion437/1
  Demux3/2 -> Data Type Conversion434/1
  Demux3/4 -> Data Type Conversion440/1
  Demux3/1 -> Data Type Conversion431/1
  Demux3/5 -> Data Type Conversion443/1
  Demux3/6 -> Data Type Conversion446/1
  Demux3/7 -> Data Type Conversion449/1
  Demux3/8 -> Data Type Conversion452/1
  Demux4/8 -> Data Type Conversion476/1
  Demux4/7 -> Data Type Conversion473/1
  Demux4/6 -> Data Type Conversion470/1
  Demux4/5 -> Data Type Conversion467/1
  Demux4/1 -> Data Type Conversion455/1
  Demux4/4 -> Data Type Conversion464/1
  Demux4/2 -> Data Type Conversion458/1
  Demux4/3 -> Data Type Conversion461/1
  Bitwise AND216/1 -> Data Type Conversion468/1
  Bitwise AND217/1 -> Shift Arithmetic150/1
  Data Type Conversion467/1 -> Bitwise AND216/1, Bitwise AND217/1
  Data Type Conversion469/1 -> Mux1/146
  Data Type Conversion468/1 -> Mux1/145
  Shift Arithmetic150/1 -> Data Type Conversion469/1
  Shift Arithmetic151/1 -> Data Type Conversion472/1
  Data Type Conversion471/1 -> Mux1/147
  Data Type Conversion472/1 -> Mux1/148
  Data Type Conversion470/1 -> Bitwise AND219/1, Bitwise AND218/1
  Bitwise AND219/1 -> Shift Arithmetic151/1
  Bitwise AND218/1 -> Data Type Conversion471/1
  Bitwise AND222/1 -> Data Type Conversion477/1
  Bitwise AND223/1 -> Shift Arithmetic153/1
  Data Type Conversion476/1 -> Bitwise AND222/1, Bitwise AND223/1
  Data Type Conversion478/1 -> Mux1/152
  Data Type Conversion477/1 -> Mux1/151
  Shift Arithmetic153/1 -> Data Type Conversion478/1
  Shift Arithmetic152/1 -> Data Type Conversion475/1
  Data Type Conversion474/1 -> Mux1/149
  Data Type Conversion475/1 -> Mux1/150
  Data Type Conversion473/1 -> Bitwise AND221/1, Bitwise AND220/1
  Bitwise AND221/1 -> Shift Arithmetic152/1
  Bitwise AND220/1 -> Data Type Conversion474/1
  Bitwise AND212/1 -> Data Type Conversion462/1
  Bitwise AND213/1 -> Shift Arithmetic148/1
  Data Type Conversion461/1 -> Bitwise AND212/1, Bitwise AND213/1
  Data Type Conversion463/1 -> Mux1/142
  Data Type Conversion462/1 -> Mux1/141
  Shift Arithmetic148/1 -> Data Type Conversion463/1
  Shift Arithmetic149/1 -> Data Type Conversion466/1
  Data Type Conversion465/1 -> Mux1/143
  Data Type Conversion466/1 -> Mux1/144
  Data Type Conversion464/1 -> Bitwise AND215/1, Bitwise AND214/1
  Bitwise AND215/1 -> Shift Arithmetic149/1
  Bitwise AND214/1 -> Data Type Conversion465/1
  Bitwise AND210/1 -> Data Type Conversion459/1
  Bitwise AND211/1 -> Shift Arithmetic147/1
  Data Type Conversion458/1 -> Bitwise AND210/1, Bitwise AND211/1
  Data Type Conversion460/1 -> Mux1/140
  Data Type Conversion459/1 -> Mux1/139
  Shift Arithmetic147/1 -> Data Type Conversion460/1
  Shift Arithmetic146/1 -> Data Type Conversion457/1
  Data Type Conversion456/1 -> Mux1/137
  Data Type Conversion457/1 -> Mux1/138
  Data Type Conversion455/1 -> Bitwise AND209/1, Bitwise AND208/1
  Bitwise AND209/1 -> Shift Arithmetic146/1
  Bitwise AND208/1 -> Data Type Conversion456/1
  VOUTP_RESSCNTDODRNGL_cnt/1 -> Demux4/1
  VOUTP_ETMATOER_kWh/1 -> Data Type Conversion479/1
  Bitwise AND227/1 -> Shift Arithmetic155/1
  Shift Arithmetic156/1 -> Data Type Conversion482/1
  Shift Arithmetic154/1 -> Data Type Conversion483/1
  Bitwise AND226/1 -> Shift Arithmetic154/1
  Bitwise AND225/1 -> Shift Arithmetic156/1
  Bitwise AND224/1 -> Data Type Conversion481/1
  Shift Arithmetic155/1 -> Data Type Conversion480/1
  Data Type Conversion479/1 -> Bitwise AND225/1, Bitwise AND226/1, Bitwise AND227/1, Bitwise AND224/1
  Data Type Conversion481/1 -> Mux1/153
  Data Type Conversion482/1 -> Mux1/154
  Data Type Conversion483/1 -> Mux1/155
  Data Type Conversion480/1 -> Mux1/156
  Data Type Conversion485/1 -> Mux1/160
  Data Type Conversion488/1 -> Mux1/159
  Data Type Conversion487/1 -> Mux1/158
  Data Type Conversion486/1 -> Mux1/157
  Data Type Conversion484/1 -> Bitwise AND228/1, Bitwise AND231/1, Bitwise AND230/1, Bitwise AND229/1
  Shift Arithmetic158/1 -> Data Type Conversion485/1
  Bitwise AND228/1 -> Data Type Conversion486/1
  Bitwise AND229/1 -> Shift Arithmetic159/1
  Bitwise AND230/1 -> Shift Arithmetic157/1
  Shift Arithmetic157/1 -> Data Type Conversion488/1
  Shift Arithmetic159/1 -> Data Type Conversion487/1
  Bitwise AND231/1 -> Shift Arithmetic158/1
  VOUTP_ETMATOEL_kWh/1 -> Data Type Conversion484/1
  VOUTP_ETMBTOEL_kWh/1 -> Data Type Conversion494/1
  Bitwise AND239/1 -> Shift Arithmetic164/1
  Shift Arithmetic165/1 -> Data Type Conversion497/1
  Shift Arithmetic163/1 -> Data Type Conversion498/1
  Bitwise AND238/1 -> Shift Arithmetic163/1
  Bitwise AND237/1 -> Shift Arithmetic165/1
  Bitwise AND236/1 -> Data Type Conversion496/1
  Shift Arithmetic164/1 -> Data Type Conversion495/1
  Data Type Conversion494/1 -> Bitwise AND237/1, Bitwise AND238/1, Bitwise AND239/1, Bitwise AND236/1
  Data Type Conversion496/1 -> Mux1/165
  Data Type Conversion497/1 -> Mux1/166
  Data Type Conversion498/1 -> Mux1/167
  Data Type Conversion495/1 -> Mux1/168
  Data Type Conversion490/1 -> Mux1/164
  Data Type Conversion493/1 -> Mux1/163
  Data Type Conversion492/1 -> Mux1/162
  Data Type Conversion491/1 -> Mux1/161
  Data Type Conversion489/1 -> Bitwise AND232/1, Bitwise AND235/1, Bitwise AND234/1, Bitwise AND233/1
  Shift Arithmetic161/1 -> Data Type Conversion490/1
  Bitwise AND232/1 -> Data Type Conversion491/1
  Bitwise AND233/1 -> Shift Arithmetic162/1
  Bitwise AND234/1 -> Shift Arithmetic160/1
  Shift Arithmetic160/1 -> Data Type Conversion493/1
  Shift Arithmetic162/1 -> Data Type Conversion492/1
  Bitwise AND235/1 -> Shift Arithmetic161/1
  VOUTP_ETMBTOER_kWh/1 -> Data Type Conversion489/1
  Bitwise AND251/1 -> Shift Arithmetic173/1
  Shift Arithmetic174/1 -> Data Type Conversion512/1
  Shift Arithmetic172/1 -> Data Type Conversion513/1
  Bitwise AND250/1 -> Shift Arithmetic172/1
  Bitwise AND249/1 -> Shift Arithmetic174/1
  Bitwise AND248/1 -> Data Type Conversion511/1
  Shift Arithmetic173/1 -> Data Type Conversion510/1
  Data Type Conversion509/1 -> Bitwise AND249/1, Bitwise AND250/1, Bitwise AND251/1, Bitwise AND248/1
  Data Type Conversion511/1 -> Mux1/177
  Data Type Conversion512/1 -> Mux1/178
  Data Type Conversion513/1 -> Mux1/179
  Data Type Conversion510/1 -> Mux1/180
  Data Type Conversion515/1 -> Mux1/184
  Data Type Conversion518/1 -> Mux1/183
  Data Type Conversion517/1 -> Mux1/182
  Data Type Conversion516/1 -> Mux1/181
  Data Type Conversion514/1 -> Bitwise AND252/1, Bitwise AND255/1, Bitwise AND254/1, Bitwise AND253/1
  Shift Arithmetic176/1 -> Data Type Conversion515/1
  Bitwise AND252/1 -> Data Type Conversion516/1
  Bitwise AND253/1 -> Shift Arithmetic177/1
  Bitwise AND254/1 -> Shift Arithmetic175/1
  Shift Arithmetic175/1 -> Data Type Conversion518/1
  Shift Arithmetic177/1 -> Data Type Conversion517/1
  Bitwise AND255/1 -> Shift Arithmetic176/1
  Bitwise AND247/1 -> Shift Arithmetic170/1
  Shift Arithmetic171/1 -> Data Type Conversion507/1
  Shift Arithmetic169/1 -> Data Type Conversion508/1
  Bitwise AND246/1 -> Shift Arithmetic169/1
  Bitwise AND245/1 -> Shift Arithmetic171/1
  Bitwise AND244/1 -> Data Type Conversion506/1
  Shift Arithmetic170/1 -> Data Type Conversion505/1
  Data Type Conversion504/1 -> Bitwise AND245/1, Bitwise AND246/1, Bitwise AND247/1, Bitwise AND244/1
  Data Type Conversion506/1 -> Mux1/173
  Data Type Conversion507/1 -> Mux1/174
  Data Type Conversion508/1 -> Mux1/175
  Data Type Conversion505/1 -> Mux1/176
  Data Type Conversion500/1 -> Mux1/172
  Data Type Conversion503/1 -> Mux1/171
  Data Type Conversion502/1 -> Mux1/170
  Data Type Conversion501/1 -> Mux1/169
  Data Type Conversion499/1 -> Bitwise AND240/1, Bitwise AND243/1, Bitwise AND242/1, Bitwise AND241/1
  Shift Arithmetic167/1 -> Data Type Conversion500/1
  Bitwise AND240/1 -> Data Type Conversion501/1
  Bitwise AND241/1 -> Shift Arithmetic168/1
  Bitwise AND242/1 -> Shift Arithmetic166/1
  Shift Arithmetic166/1 -> Data Type Conversion503/1
  Shift Arithmetic168/1 -> Data Type Conversion502/1
  Bitwise AND243/1 -> Shift Arithmetic167/1
  Bitwise AND259/1 -> Shift Arithmetic179/1
  Shift Arithmetic180/1 -> Data Type Conversion522/1
  Shift Arithmetic178/1 -> Data Type Conversion523/1
  Bitwise AND258/1 -> Shift Arithmetic178/1
  Bitwise AND257/1 -> Shift Arithmetic180/1
  Bitwise AND256/1 -> Data Type Conversion521/1
  Shift Arithmetic179/1 -> Data Type Conversion520/1
  Data Type Conversion519/1 -> Bitwise AND257/1, Bitwise AND258/1, Bitwise AND259/1, Bitwise AND256/1
  Data Type Conversion521/1 -> Mux1/185
  Data Type Conversion522/1 -> Mux1/186
  Data Type Conversion523/1 -> Mux1/187
  Data Type Conversion520/1 -> Mux1/188
  Data Type Conversion525/1 -> Mux1/192
  Data Type Conversion528/1 -> Mux1/191
  Data Type Conversion527/1 -> Mux1/190
  Data Type Conversion526/1 -> Mux1/189
  Data Type Conversion524/1 -> Bitwise AND260/1, Bitwise AND263/1, Bitwise AND262/1, Bitwise AND261/1
  Shift Arithmetic182/1 -> Data Type Conversion525/1
  Bitwise AND260/1 -> Data Type Conversion526/1
  Bitwise AND261/1 -> Shift Arithmetic183/1
  Bitwise AND262/1 -> Shift Arithmetic181/1
  Shift Arithmetic181/1 -> Data Type Conversion528/1
  Shift Arithmetic183/1 -> Data Type Conversion527/1
  Bitwise AND263/1 -> Shift Arithmetic182/1
  Bitwise AND271/1 -> Shift Arithmetic188/1
  Shift Arithmetic189/1 -> Data Type Conversion537/1
  Shift Arithmetic187/1 -> Data Type Conversion538/1
  Bitwise AND270/1 -> Shift Arithmetic187/1
  Bitwise AND269/1 -> Shift Arithmetic189/1
  Bitwise AND268/1 -> Data Type Conversion536/1
  Shift Arithmetic188/1 -> Data Type Conversion535/1
  Data Type Conversion534/1 -> Bitwise AND269/1, Bitwise AND270/1, Bitwise AND271/1, Bitwise AND268/1
  Data Type Conversion536/1 -> Mux1/197
  Data Type Conversion537/1 -> Mux1/198
  Data Type Conversion538/1 -> Mux1/199
  Data Type Conversion535/1 -> Mux1/200
  Data Type Conversion530/1 -> Mux1/196
  Data Type Conversion533/1 -> Mux1/195
  Data Type Conversion532/1 -> Mux1/194
  Data Type Conversion531/1 -> Mux1/193
  Data Type Conversion529/1 -> Bitwise AND264/1, Bitwise AND267/1, Bitwise AND266/1, Bitwise AND265/1
  Shift Arithmetic185/1 -> Data Type Conversion530/1
  Bitwise AND264/1 -> Data Type Conversion531/1
  Bitwise AND265/1 -> Shift Arithmetic186/1
  Bitwise AND266/1 -> Shift Arithmetic184/1
  Shift Arithmetic184/1 -> Data Type Conversion533/1
  Shift Arithmetic186/1 -> Data Type Conversion532/1
  Bitwise AND267/1 -> Shift Arithmetic185/1
  Demux5/1 -> Data Type Conversion499/1
  Demux5/2 -> Data Type Conversion504/1
  Demux5/3 -> Data Type Conversion509/1
  Demux5/4 -> Data Type Conversion514/1
  Demux5/5 -> Data Type Conversion519/1
  Demux5/6 -> Data Type Conversion524/1
  Demux5/7 -> Data Type Conversion529/1
  Demux5/8 -> Data Type Conversion534/1
  VOUTP_RESSTIMESOCPSARNGR_s/1 -> Demux5/1
  VOUTP_RESSTIMESOCPSARNGL_s/1 -> Demux6/1
  Demux6/8 -> Data Type Conversion574/1
  Demux6/7 -> Data Type Conversion569/1
  Demux6/6 -> Data Type Conversion564/1
  Demux6/5 -> Data Type Conversion559/1
  Demux6/4 -> Data Type Conversion554/1
  Demux6/3 -> Data Type Conversion549/1
  Demux6/2 -> Data Type Conversion544/1
  Demux6/1 -> Data Type Conversion539/1
  Bitwise AND299/1 -> Shift Arithmetic209/1
  Shift Arithmetic210/1 -> Data Type Conversion572/1
  Shift Arithmetic208/1 -> Data Type Conversion573/1
  Bitwise AND298/1 -> Shift Arithmetic208/1
  Bitwise AND297/1 -> Shift Arithmetic210/1
  Bitwise AND296/1 -> Data Type Conversion571/1
  Shift Arithmetic209/1 -> Data Type Conversion570/1
  Data Type Conversion569/1 -> Bitwise AND297/1, Bitwise AND298/1, Bitwise AND299/1, Bitwise AND296/1
  Data Type Conversion571/1 -> Mux1/225
  Data Type Conversion572/1 -> Mux1/226
  Data Type Conversion573/1 -> Mux1/227
  Data Type Conversion570/1 -> Mux1/228
  Data Type Conversion575/1 -> Mux1/232
  Data Type Conversion578/1 -> Mux1/231
  Data Type Conversion577/1 -> Mux1/230
  Data Type Conversion576/1 -> Mux1/229
  Data Type Conversion574/1 -> Bitwise AND300/1, Bitwise AND303/1, Bitwise AND302/1, Bitwise AND301/1
  Shift Arithmetic212/1 -> Data Type Conversion575/1
  Bitwise AND300/1 -> Data Type Conversion576/1
  Bitwise AND301/1 -> Shift Arithmetic213/1
  Bitwise AND302/1 -> Shift Arithmetic211/1
  Shift Arithmetic211/1 -> Data Type Conversion578/1
  Shift Arithmetic213/1 -> Data Type Conversion577/1
  Bitwise AND303/1 -> Shift Arithmetic212/1
  Bitwise AND295/1 -> Shift Arithmetic206/1
  Shift Arithmetic207/1 -> Data Type Conversion567/1
  Shift Arithmetic205/1 -> Data Type Conversion568/1
  Bitwise AND294/1 -> Shift Arithmetic205/1
  Bitwise AND293/1 -> Shift Arithmetic207/1
  Bitwise AND292/1 -> Data Type Conversion566/1
  Shift Arithmetic206/1 -> Data Type Conversion565/1
  Data Type Conversion564/1 -> Bitwise AND293/1, Bitwise AND294/1, Bitwise AND295/1, Bitwise AND292/1
  Data Type Conversion566/1 -> Mux1/221
  Data Type Conversion567/1 -> Mux1/222
  Data Type Conversion568/1 -> Mux1/223
  Data Type Conversion565/1 -> Mux1/224
  Data Type Conversion560/1 -> Mux1/220
  Data Type Conversion563/1 -> Mux1/219
  Data Type Conversion562/1 -> Mux1/218
  Data Type Conversion561/1 -> Mux1/217
  Data Type Conversion559/1 -> Bitwise AND288/1, Bitwise AND291/1, Bitwise AND290/1, Bitwise AND289/1
  Shift Arithmetic203/1 -> Data Type Conversion560/1
  Bitwise AND288/1 -> Data Type Conversion561/1
  Bitwise AND289/1 -> Shift Arithmetic204/1
  Bitwise AND290/1 -> Shift Arithmetic202/1
  Shift Arithmetic202/1 -> Data Type Conversion563/1
  Shift Arithmetic204/1 -> Data Type Conversion562/1
  Bitwise AND291/1 -> Shift Arithmetic203/1
  Bitwise AND275/1 -> Shift Arithmetic191/1
  Shift Arithmetic192/1 -> Data Type Conversion542/1
  Shift Arithmetic190/1 -> Data Type Conversion543/1
  Bitwise AND274/1 -> Shift Arithmetic190/1
  Bitwise AND273/1 -> Shift Arithmetic192/1
  Bitwise AND272/1 -> Data Type Conversion541/1
  Shift Arithmetic191/1 -> Data Type Conversion540/1
  Data Type Conversion539/1 -> Bitwise AND273/1, Bitwise AND274/1, Bitwise AND275/1, Bitwise AND272/1
  Data Type Conversion541/1 -> Mux1/201
  Data Type Conversion542/1 -> Mux1/202
  Data Type Conversion543/1 -> Mux1/203
  Data Type Conversion540/1 -> Mux1/204
  Data Type Conversion545/1 -> Mux1/208
  Data Type Conversion548/1 -> Mux1/207
  Data Type Conversion547/1 -> Mux1/206
  Data Type Conversion546/1 -> Mux1/205
  Data Type Conversion544/1 -> Bitwise AND276/1, Bitwise AND279/1, Bitwise AND278/1, Bitwise AND277/1
  Shift Arithmetic194/1 -> Data Type Conversion545/1
  Bitwise AND276/1 -> Data Type Conversion546/1
  Bitwise AND277/1 -> Shift Arithmetic195/1
  Bitwise AND278/1 -> Shift Arithmetic193/1
  Shift Arithmetic193/1 -> Data Type Conversion548/1
  Shift Arithmetic195/1 -> Data Type Conversion547/1
  Bitwise AND279/1 -> Shift Arithmetic194/1
  Bitwise AND287/1 -> Shift Arithmetic200/1
  Shift Arithmetic201/1 -> Data Type Conversion557/1
  Shift Arithmetic199/1 -> Data Type Conversion558/1
  Bitwise AND286/1 -> Shift Arithmetic199/1
  Bitwise AND285/1 -> Shift Arithmetic201/1
  Bitwise AND284/1 -> Data Type Conversion556/1
  Shift Arithmetic200/1 -> Data Type Conversion555/1
  Data Type Conversion554/1 -> Bitwise AND285/1, Bitwise AND286/1, Bitwise AND287/1, Bitwise AND284/1
  Data Type Conversion556/1 -> Mux1/213
  Data Type Conversion557/1 -> Mux1/214
  Data Type Conversion558/1 -> Mux1/215
  Data Type Conversion555/1 -> Mux1/216
  Data Type Conversion550/1 -> Mux1/212
  Data Type Conversion553/1 -> Mux1/211
  Data Type Conversion552/1 -> Mux1/210
  Data Type Conversion551/1 -> Mux1/209
  Data Type Conversion549/1 -> Bitwise AND280/1, Bitwise AND283/1, Bitwise AND282/1, Bitwise AND281/1
  Shift Arithmetic197/1 -> Data Type Conversion550/1
  Bitwise AND280/1 -> Data Type Conversion551/1
  Bitwise AND281/1 -> Shift Arithmetic198/1
  Bitwise AND282/1 -> Shift Arithmetic196/1
  Shift Arithmetic196/1 -> Data Type Conversion553/1
  Shift Arithmetic198/1 -> Data Type Conversion552/1
  Bitwise AND283/1 -> Shift Arithmetic197/1
  VOUTP_RESSTIMESOCCHGRNGR_s/1 -> Demux7/1
  Demux7/8 -> [VOUTP_RESSTIMESOCCHGRNGR7_s]
  Demux7/7 -> [VOUTP_RESSTIMESOCCHGRNGR67_s]
  Demux7/6 -> Data Type Conversion604/1
  Demux7/5 -> Data Type Conversion599/1
  Demux7/4 -> Data Type Conversion594/1
  Demux7/3 -> Data Type Conversion589/1
  Demux7/2 -> Data Type Conversion584/1
  Demux7/1 -> Data Type Conversion579/1
  Bitwise AND327/1 -> Shift Arithmetic230/1
  Shift Arithmetic231/1 -> Data Type Conversion607/1
  Shift Arithmetic229/1 -> Data Type Conversion608/1
  Bitwise AND326/1 -> Shift Arithmetic229/1
  Bitwise AND325/1 -> Shift Arithmetic231/1
  Bitwise AND324/1 -> Data Type Conversion606/1
  Shift Arithmetic230/1 -> Data Type Conversion605/1
  Data Type Conversion604/1 -> Bitwise AND325/1, Bitwise AND326/1, Bitwise AND327/1, Bitwise AND324/1
  Data Type Conversion606/1 -> Mux1/253
  Data Type Conversion607/1 -> Mux1/254
  Data Type Conversion608/1 -> Mux1/255
  Data Type Conversion605/1 -> Mux1/256
  Data Type Conversion600/1 -> Mux1/252
  Data Type Conversion603/1 -> Mux1/251
  Data Type Conversion602/1 -> Mux1/250
  Data Type Conversion601/1 -> Mux1/249
  Data Type Conversion599/1 -> Bitwise AND320/1, Bitwise AND323/1, Bitwise AND322/1, Bitwise AND321/1
  Shift Arithmetic227/1 -> Data Type Conversion600/1
  Bitwise AND320/1 -> Data Type Conversion601/1
  Bitwise AND321/1 -> Shift Arithmetic228/1
  Bitwise AND322/1 -> Shift Arithmetic226/1
  Shift Arithmetic226/1 -> Data Type Conversion603/1
  Shift Arithmetic228/1 -> Data Type Conversion602/1
  Bitwise AND323/1 -> Shift Arithmetic227/1
  Bitwise AND307/1 -> Shift Arithmetic215/1
  Shift Arithmetic216/1 -> Data Type Conversion582/1
  Shift Arithmetic214/1 -> Data Type Conversion583/1
  Bitwise AND306/1 -> Shift Arithmetic214/1
  Bitwise AND305/1 -> Shift Arithmetic216/1
  Bitwise AND304/1 -> Data Type Conversion581/1
  Shift Arithmetic215/1 -> Data Type Conversion580/1
  Data Type Conversion579/1 -> Bitwise AND305/1, Bitwise AND306/1, Bitwise AND307/1, Bitwise AND304/1
  Data Type Conversion581/1 -> Mux1/233
  Data Type Conversion582/1 -> Mux1/234
  Data Type Conversion583/1 -> Mux1/235
  Data Type Conversion580/1 -> Mux1/236
  Data Type Conversion585/1 -> Mux1/240
  Data Type Conversion588/1 -> Mux1/239
  Data Type Conversion587/1 -> Mux1/238
  Data Type Conversion586/1 -> Mux1/237
  Data Type Conversion584/1 -> Bitwise AND308/1, Bitwise AND311/1, Bitwise AND310/1, Bitwise AND309/1
  Shift Arithmetic218/1 -> Data Type Conversion585/1
  Bitwise AND308/1 -> Data Type Conversion586/1
  Bitwise AND309/1 -> Shift Arithmetic219/1
  Bitwise AND310/1 -> Shift Arithmetic217/1
  Shift Arithmetic217/1 -> Data Type Conversion588/1
  Shift Arithmetic219/1 -> Data Type Conversion587/1
  Bitwise AND311/1 -> Shift Arithmetic218/1
  Bitwise AND319/1 -> Shift Arithmetic224/1
  Shift Arithmetic225/1 -> Data Type Conversion597/1
  Shift Arithmetic223/1 -> Data Type Conversion598/1
  Bitwise AND318/1 -> Shift Arithmetic223/1
  Bitwise AND317/1 -> Shift Arithmetic225/1
  Bitwise AND316/1 -> Data Type Conversion596/1
  Shift Arithmetic224/1 -> Data Type Conversion595/1
  Data Type Conversion594/1 -> Bitwise AND317/1, Bitwise AND318/1, Bitwise AND319/1, Bitwise AND316/1
  Data Type Conversion596/1 -> Mux1/245
  Data Type Conversion597/1 -> Mux1/246
  Data Type Conversion598/1 -> Mux1/247
  Data Type Conversion595/1 -> Mux1/248
  Data Type Conversion590/1 -> Mux1/244
  Data Type Conversion593/1 -> Mux1/243
  Data Type Conversion592/1 -> Mux1/242
  Data Type Conversion591/1 -> Mux1/241
  Data Type Conversion589/1 -> Bitwise AND312/1, Bitwise AND315/1, Bitwise AND314/1, Bitwise AND313/1
  Shift Arithmetic221/1 -> Data Type Conversion590/1
  Bitwise AND312/1 -> Data Type Conversion591/1
  Bitwise AND313/1 -> Shift Arithmetic222/1
  Bitwise AND314/1 -> Shift Arithmetic220/1
  Shift Arithmetic220/1 -> Data Type Conversion593/1
  Shift Arithmetic222/1 -> Data Type Conversion592/1
  Bitwise AND315/1 -> Shift Arithmetic221/1
  Bitwise AND334/1 -> Shift Arithmetic235/1
  Shift Arithmetic237/1 -> Data Type Conversion617/1
  Shift Arithmetic235/1 -> Data Type Conversion618/1
  Shift Arithmetic236/1 -> Data Type Conversion615/1
  Bitwise AND332/1 -> Data Type Conversion616/1
  Data Type Conversion614/1 -> Bitwise AND332/1, Bitwise AND335/1, Bitwise AND334/1, Bitwise AND333/1
  Data Type Conversion617/1 -> Mux3/6
  Data Type Conversion616/1 -> Mux3/5
  Data Type Conversion618/1 -> Mux3/7
  Data Type Conversion610/1 -> Mux3/4
  Data Type Conversion611/1 -> Mux3/1
  Data Type Conversion612/1 -> Mux3/2
  Data Type Conversion609/1 -> Bitwise AND329/1, Bitwise AND330/1, Bitwise AND331/1, Bitwise AND328/1
  Bitwise AND333/1 -> Shift Arithmetic237/1
  Data Type Conversion615/1 -> Mux3/8
  Bitwise AND328/1 -> Data Type Conversion611/1
  Shift Arithmetic233/1 -> Data Type Conversion610/1
  Data Type Conversion613/1 -> Mux3/3
  [VOUTP_RESSTIMESOCCHGRNGR7_s] -> Data Type Conversion614/1
  Bitwise AND331/1 -> Shift Arithmetic233/1
  Shift Arithmetic234/1 -> Data Type Conversion612/1
  Bitwise AND330/1 -> Shift Arithmetic232/1
  Shift Arithmetic232/1 -> Data Type Conversion613/1
  Bitwise AND335/1 -> Shift Arithmetic236/1
  [VOUTP_RESSTIMESOCCHGRNGR67_s] -> Data Type Conversion609/1
  Bitwise AND329/1 -> Shift Arithmetic234/1
  Bitwise AND344/1 -> Data Type Conversion631/1
  Data Type Conversion629/1 -> Bitwise AND345/1, Bitwise AND346/1, Bitwise AND347/1, Bitwise AND344/1
  Bitwise AND345/1 -> Shift Arithmetic246/1
  Shift Arithmetic245/1 -> Data Type Conversion630/1
  Bitwise AND346/1 -> Shift Arithmetic244/1
  Shift Arithmetic244/1 -> Data Type Conversion633/1
  Shift Arithmetic246/1 -> Data Type Conversion632/1
  Bitwise AND347/1 -> Shift Arithmetic245/1
  Data Type Conversion634/1 -> Bitwise AND348/1, Bitwise AND351/1, Bitwise AND350/1, Bitwise AND349/1
  Shift Arithmetic248/1 -> Data Type Conversion635/1
  Bitwise AND350/1 -> Shift Arithmetic247/1
  Bitwise AND349/1 -> Shift Arithmetic249/1
  Bitwise AND348/1 -> Data Type Conversion636/1
  Data Type Conversion658/1 -> Mux3/39
  Data Type Conversion642/1 -> Mux3/26
  Data Type Conversion656/1 -> Mux3/37
  Data Type Conversion645/1 -> Mux3/32
  Data Type Conversion657/1 -> Mux3/38
  Data Type Conversion646/1 -> Mux3/29
  Data Type Conversion652/1 -> Mux3/34
  Data Type Conversion640/1 -> Mux3/28
  Data Type Conversion653/1 -> Mux3/35
  Data Type Conversion643/1 -> Mux3/27
  Data Type Conversion655/1 -> Mux3/40
  Data Type Conversion650/1 -> Mux3/36
  Data Type Conversion641/1 -> Mux3/25
  Data Type Conversion628/1 -> Mux3/15
  Data Type Conversion651/1 -> Mux3/33
  Data Type Conversion625/1 -> Mux3/16
  Data Type Conversion637/1 -> Mux3/22
  Data Type Conversion632/1 -> Mux3/18
  Data Type Conversion626/1 -> Mux3/13
  Data Type Conversion620/1 -> Mux3/12
  Data Type Conversion633/1 -> Mux3/19
  Data Type Conversion622/1 -> Mux3/10
  Data Type Conversion627/1 -> Mux3/14
  Data Type Conversion638/1 -> Mux3/23
  Bitwise AND362/1 -> Shift Arithmetic256/1
  Data Type Conversion636/1 -> Mux3/21
  Data Type Conversion649/1 -> Bitwise AND360/1, Bitwise AND363/1, Bitwise AND362/1, Bitwise AND361/1
  Shift Arithmetic257/1 -> Data Type Conversion650/1
  Bitwise AND360/1 -> Data Type Conversion651/1
  Data Type Conversion647/1 -> Mux3/30
  Bitwise AND364/1 -> Data Type Conversion656/1
  Data Type Conversion631/1 -> Mux3/17
  Bitwise AND365/1 -> Shift Arithmetic261/1
  Shift Arithmetic260/1 -> Data Type Conversion655/1
  Data Type Conversion654/1 -> Bitwise AND365/1, Bitwise AND366/1, Bitwise AND367/1, Bitwise AND364/1
  Data Type Conversion623/1 -> Mux3/11
  Shift Arithmetic259/1 -> Data Type Conversion658/1
  Shift Arithmetic253/1 -> Data Type Conversion648/1
  Shift Arithmetic254/1 -> Data Type Conversion645/1
  Bitwise AND356/1 -> Data Type Conversion646/1
  Shift Arithmetic255/1 -> Data Type Conversion647/1
  Data Type Conversion644/1 -> Bitwise AND356/1, Bitwise AND359/1, Bitwise AND358/1, Bitwise AND357/1
  Shift Arithmetic261/1 -> Data Type Conversion657/1
  Bitwise AND367/1 -> Shift Arithmetic260/1
  Bitwise AND359/1 -> Shift Arithmetic254/1
  Bitwise AND357/1 -> Shift Arithmetic255/1
  Bitwise AND358/1 -> Shift Arithmetic253/1
  Data Type Conversion639/1 -> Bitwise AND353/1, Bitwise AND354/1, Bitwise AND355/1, Bitwise AND352/1
  Bitwise AND354/1 -> Shift Arithmetic250/1
  Shift Arithmetic250/1 -> Data Type Conversion643/1
  Bitwise AND352/1 -> Data Type Conversion641/1
  Bitwise AND355/1 -> Shift Arithmetic251/1
  Shift Arithmetic256/1 -> Data Type Conversion653/1
  Demux8/7 -> Data Type Conversion649/1
  Demux8/8 -> Data Type Conversion654/1
  Demux8/4 -> Data Type Conversion634/1
  Demux8/3 -> Data Type Conversion629/1
  Bitwise AND366/1 -> Shift Arithmetic259/1
  Demux8/5 -> Data Type Conversion639/1
  Demux8/1 -> Data Type Conversion619/1
  Data Type Conversion635/1 -> Mux3/24
  Shift Arithmetic252/1 -> Data Type Conversion642/1
  Data Type Conversion624/1 -> Bitwise AND341/1, Bitwise AND342/1, Bitwise AND343/1, Bitwise AND340/1
  Bitwise AND353/1 -> Shift Arithmetic252/1
  Bitwise AND341/1 -> Shift Arithmetic243/1
  Bitwise AND342/1 -> Shift Arithmetic241/1
  Data Type Conversion630/1 -> Mux3/20
  Shift Arithmetic242/1 -> Data Type Conversion625/1
  Bitwise AND340/1 -> Data Type Conversion626/1
  Shift Arithmetic241/1 -> Data Type Conversion628/1
  Bitwise AND351/1 -> Shift Arithmetic248/1
  Bitwise AND363/1 -> Shift Arithmetic257/1
  Bitwise AND343/1 -> Shift Arithmetic242/1
  Shift Arithmetic249/1 -> Data Type Conversion637/1
  Shift Arithmetic251/1 -> Data Type Conversion640/1
  Shift Arithmetic247/1 -> Data Type Conversion638/1
  Shift Arithmetic243/1 -> Data Type Conversion627/1
  Shift Arithmetic240/1 -> Data Type Conversion622/1
  Bitwise AND339/1 -> Shift Arithmetic239/1
  Shift Arithmetic238/1 -> Data Type Conversion623/1
  Bitwise AND336/1 -> Data Type Conversion621/1
  Demux8/6 -> Data Type Conversion644/1
  Data Type Conversion619/1 -> Bitwise AND336/1, Bitwise AND339/1, Bitwise AND338/1, Bitwise AND337/1
  Bitwise AND338/1 -> Shift Arithmetic238/1
  Bitwise AND361/1 -> Shift Arithmetic258/1
  Shift Arithmetic239/1 -> Data Type Conversion620/1
  Shift Arithmetic258/1 -> Data Type Conversion652/1
  Demux8/2 -> Data Type Conversion624/1
  Bitwise AND337/1 -> Shift Arithmetic240/1
  Data Type Conversion648/1 -> Mux3/31
  Data Type Conversion621/1 -> Mux3/9
  VOUTP_RESSTIMESOCCHGRNGL_s/1 -> Demux8/1
  VOUTP_RESSTIMESOCOFFRNGR_s/1 -> Demux9/1
  Data Type Conversion661/1 -> Mux3/41
  Data Type Conversion688/1 -> Mux3/63
  Bitwise AND369/1 -> Shift Arithmetic264/1
  Demux9/2 -> Data Type Conversion664/1
  Shift Arithmetic282/1 -> Data Type Conversion692/1
  Shift Arithmetic263/1 -> Data Type Conversion660/1
  Bitwise AND393/1 -> Shift Arithmetic282/1
  Bitwise AND370/1 -> Shift Arithmetic262/1
  Data Type Conversion659/1 -> Bitwise AND369/1, Bitwise AND370/1, Bitwise AND371/1, Bitwise AND368/1
  Demux9/6 -> Data Type Conversion684/1
  Bitwise AND368/1 -> Data Type Conversion661/1
  Shift Arithmetic262/1 -> Data Type Conversion663/1
  Bitwise AND371/1 -> Shift Arithmetic263/1
  Shift Arithmetic264/1 -> Data Type Conversion662/1
  Shift Arithmetic267/1 -> Data Type Conversion667/1
  Shift Arithmetic271/1 -> Data Type Conversion678/1
  Shift Arithmetic275/1 -> Data Type Conversion680/1
  Shift Arithmetic273/1 -> Data Type Conversion677/1
  Bitwise AND375/1 -> Shift Arithmetic266/1
  Bitwise AND395/1 -> Shift Arithmetic281/1
  Bitwise AND383/1 -> Shift Arithmetic272/1
  Shift Arithmetic265/1 -> Data Type Conversion668/1
  Bitwise AND372/1 -> Data Type Conversion666/1
  Shift Arithmetic266/1 -> Data Type Conversion665/1
  Data Type Conversion670/1 -> Mux3/52
  Bitwise AND374/1 -> Shift Arithmetic265/1
  Bitwise AND373/1 -> Shift Arithmetic267/1
  Bitwise AND385/1 -> Shift Arithmetic276/1
  Data Type Conversion664/1 -> Bitwise AND372/1, Bitwise AND375/1, Bitwise AND374/1, Bitwise AND373/1
  Shift Arithmetic276/1 -> Data Type Conversion682/1
  Data Type Conversion675/1 -> Mux3/56
  Demux9/1 -> Data Type Conversion659/1
  Demux9/5 -> Data Type Conversion679/1
  Bitwise AND398/1 -> Shift Arithmetic283/1
  Demux9/3 -> Data Type Conversion669/1
  Demux9/4 -> Data Type Conversion674/1
  Demux9/8 -> Data Type Conversion694/1
  Demux9/7 -> Data Type Conversion689/1
  Shift Arithmetic280/1 -> Data Type Conversion693/1
  Bitwise AND387/1 -> Shift Arithmetic275/1
  Bitwise AND384/1 -> Data Type Conversion681/1
  Shift Arithmetic274/1 -> Data Type Conversion683/1
  Bitwise AND386/1 -> Shift Arithmetic274/1
  Data Type Conversion679/1 -> Bitwise AND384/1, Bitwise AND387/1, Bitwise AND386/1, Bitwise AND385/1
  Bitwise AND390/1 -> Shift Arithmetic277/1
  Bitwise AND389/1 -> Shift Arithmetic279/1
  Bitwise AND391/1 -> Shift Arithmetic278/1
  Bitwise AND399/1 -> Shift Arithmetic284/1
  Shift Arithmetic285/1 -> Data Type Conversion697/1
  Data Type Conversion684/1 -> Bitwise AND389/1, Bitwise AND390/1, Bitwise AND391/1, Bitwise AND388/1
  Shift Arithmetic279/1 -> Data Type Conversion687/1
  Bitwise AND388/1 -> Data Type Conversion686/1
  Shift Arithmetic278/1 -> Data Type Conversion685/1
  Shift Arithmetic277/1 -> Data Type Conversion688/1
  Shift Arithmetic283/1 -> Data Type Conversion698/1
  Data Type Conversion663/1 -> Mux3/43
  Data Type Conversion694/1 -> Bitwise AND396/1, Bitwise AND399/1, Bitwise AND398/1, Bitwise AND397/1
  Shift Arithmetic284/1 -> Data Type Conversion695/1
  Bitwise AND397/1 -> Shift Arithmetic285/1
  Data Type Conversion671/1 -> Mux3/49
  Bitwise AND396/1 -> Data Type Conversion696/1
  Data Type Conversion687/1 -> Mux3/62
  Bitwise AND392/1 -> Data Type Conversion691/1
  Shift Arithmetic281/1 -> Data Type Conversion690/1
  Data Type Conversion689/1 -> Bitwise AND393/1, Bitwise AND394/1, Bitwise AND395/1, Bitwise AND392/1
  Data Type Conversion676/1 -> Mux3/53
  Bitwise AND394/1 -> Shift Arithmetic280/1
  Data Type Conversion678/1 -> Mux3/55
  Data Type Conversion667/1 -> Mux3/46
  Data Type Conversion662/1 -> Mux3/42
  Data Type Conversion673/1 -> Mux3/51
  Data Type Conversion660/1 -> Mux3/44
  Data Type Conversion666/1 -> Mux3/45
  Data Type Conversion672/1 -> Mux3/50
  Data Type Conversion677/1 -> Mux3/54
  Data Type Conversion665/1 -> Mux3/48
  Data Type Conversion691/1 -> Mux3/65
  Data Type Conversion668/1 -> Mux3/47
  Data Type Conversion681/1 -> Mux3/57
  Data Type Conversion690/1 -> Mux3/68
  Data Type Conversion695/1 -> Mux3/72
  Data Type Conversion683/1 -> Mux3/59
  Data Type Conversion693/1 -> Mux3/67
  Data Type Conversion680/1 -> Mux3/60
  Data Type Conversion692/1 -> Mux3/66
  Data Type Conversion686/1 -> Mux3/61
  Data Type Conversion697/1 -> Mux3/70
  Data Type Conversion685/1 -> Mux3/64
  Data Type Conversion696/1 -> Mux3/69
  Data Type Conversion682/1 -> Mux3/58
  Data Type Conversion698/1 -> Mux3/71
  Bitwise AND380/1 -> Data Type Conversion676/1
  Bitwise AND381/1 -> Shift Arithmetic273/1
  Bitwise AND382/1 -> Shift Arithmetic271/1
  Shift Arithmetic272/1 -> Data Type Conversion675/1
  Data Type Conversion674/1 -> Bitwise AND381/1, Bitwise AND382/1, Bitwise AND383/1, Bitwise AND380/1
  Bitwise AND379/1 -> Shift Arithmetic269/1
  Shift Arithmetic270/1 -> Data Type Conversion672/1
  Shift Arithmetic268/1 -> Data Type Conversion673/1
  Bitwise AND378/1 -> Shift Arithmetic268/1
  Shift Arithmetic269/1 -> Data Type Conversion670/1
  Bitwise AND377/1 -> Shift Arithmetic270/1
  Data Type Conversion669/1 -> Bitwise AND376/1, Bitwise AND379/1, Bitwise AND378/1, Bitwise AND377/1
  Bitwise AND376/1 -> Data Type Conversion671/1
  Bitwise AND408/1 -> Data Type Conversion711/1
  Data Type Conversion709/1 -> Bitwise AND409/1, Bitwise AND410/1, Bitwise AND411/1, Bitwise AND408/1
  Bitwise AND409/1 -> Shift Arithmetic294/1
  Shift Arithmetic293/1 -> Data Type Conversion710/1
  Bitwise AND410/1 -> Shift Arithmetic292/1
  Shift Arithmetic292/1 -> Data Type Conversion713/1
  Shift Arithmetic294/1 -> Data Type Conversion712/1
  Bitwise AND411/1 -> Shift Arithmetic293/1
  Data Type Conversion714/1 -> Bitwise AND412/1, Bitwise AND415/1, Bitwise AND414/1, Bitwise AND413/1
  Shift Arithmetic296/1 -> Data Type Conversion715/1
  Bitwise AND414/1 -> Shift Arithmetic295/1
  Bitwise AND413/1 -> Shift Arithmetic297/1
  Bitwise AND412/1 -> Data Type Conversion716/1
  Data Type Conversion738/1 -> Mux3/103
  Data Type Conversion722/1 -> Mux3/90
  Data Type Conversion736/1 -> Mux3/101
  Data Type Conversion725/1 -> Mux3/96
  Data Type Conversion737/1 -> Mux3/102
  Data Type Conversion726/1 -> Mux3/93
  Data Type Conversion732/1 -> Mux3/98
  Data Type Conversion720/1 -> Mux3/92
  Data Type Conversion733/1 -> Mux3/99
  Data Type Conversion723/1 -> Mux3/91
  Data Type Conversion735/1 -> Mux3/104
  Data Type Conversion730/1 -> Mux3/100
  Data Type Conversion721/1 -> Mux3/89
  Data Type Conversion708/1 -> Mux3/79
  Data Type Conversion731/1 -> Mux3/97
  Data Type Conversion705/1 -> Mux3/80
  Data Type Conversion717/1 -> Mux3/86
  Data Type Conversion712/1 -> Mux3/82
  Data Type Conversion706/1 -> Mux3/77
  Data Type Conversion700/1 -> Mux3/76
  Data Type Conversion713/1 -> Mux3/83
  Data Type Conversion702/1 -> Mux3/74
  Data Type Conversion707/1 -> Mux3/78
  Data Type Conversion718/1 -> Mux3/87
  Bitwise AND426/1 -> Shift Arithmetic304/1
  Data Type Conversion716/1 -> Mux3/85
  Data Type Conversion729/1 -> Bitwise AND424/1, Bitwise AND427/1, Bitwise AND426/1, Bitwise AND425/1
  Shift Arithmetic305/1 -> Data Type Conversion730/1
  Bitwise AND424/1 -> Data Type Conversion731/1
  Data Type Conversion727/1 -> Mux3/94
  Bitwise AND428/1 -> Data Type Conversion736/1
  Data Type Conversion711/1 -> Mux3/81
  Bitwise AND429/1 -> Shift Arithmetic309/1
  Shift Arithmetic308/1 -> Data Type Conversion735/1
  Data Type Conversion734/1 -> Bitwise AND429/1, Bitwise AND430/1, Bitwise AND431/1, Bitwise AND428/1
  Data Type Conversion703/1 -> Mux3/75
  Shift Arithmetic307/1 -> Data Type Conversion738/1
  Shift Arithmetic301/1 -> Data Type Conversion728/1
  Shift Arithmetic302/1 -> Data Type Conversion725/1
  Bitwise AND420/1 -> Data Type Conversion726/1
  Shift Arithmetic303/1 -> Data Type Conversion727/1
  Data Type Conversion724/1 -> Bitwise AND420/1, Bitwise AND423/1, Bitwise AND422/1, Bitwise AND421/1
  Shift Arithmetic309/1 -> Data Type Conversion737/1
  Bitwise AND431/1 -> Shift Arithmetic308/1
  Bitwise AND423/1 -> Shift Arithmetic302/1
  Bitwise AND421/1 -> Shift Arithmetic303/1
  Bitwise AND422/1 -> Shift Arithmetic301/1
  Data Type Conversion719/1 -> Bitwise AND417/1, Bitwise AND418/1, Bitwise AND419/1, Bitwise AND416/1
  Bitwise AND418/1 -> Shift Arithmetic298/1
  Shift Arithmetic298/1 -> Data Type Conversion723/1
  Bitwise AND416/1 -> Data Type Conversion721/1
  Bitwise AND419/1 -> Shift Arithmetic299/1
  Shift Arithmetic304/1 -> Data Type Conversion733/1
  Demux10/7 -> Data Type Conversion729/1
  Demux10/8 -> Data Type Conversion734/1
  Demux10/4 -> Data Type Conversion714/1
  Demux10/3 -> Data Type Conversion709/1
  Bitwise AND430/1 -> Shift Arithmetic307/1
  Demux10/5 -> Data Type Conversion719/1
  Demux10/1 -> Data Type Conversion699/1
  Data Type Conversion715/1 -> Mux3/88
  Shift Arithmetic300/1 -> Data Type Conversion722/1
  Data Type Conversion704/1 -> Bitwise AND405/1, Bitwise AND406/1, Bitwise AND407/1, Bitwise AND404/1
  Bitwise AND417/1 -> Shift Arithmetic300/1
  Bitwise AND405/1 -> Shift Arithmetic291/1
  Bitwise AND406/1 -> Shift Arithmetic289/1
  Data Type Conversion710/1 -> Mux3/84
  Shift Arithmetic290/1 -> Data Type Conversion705/1
  Bitwise AND404/1 -> Data Type Conversion706/1
  Shift Arithmetic289/1 -> Data Type Conversion708/1
  Bitwise AND415/1 -> Shift Arithmetic296/1
  Bitwise AND427/1 -> Shift Arithmetic305/1
  Bitwise AND407/1 -> Shift Arithmetic290/1
  Shift Arithmetic297/1 -> Data Type Conversion717/1
  Shift Arithmetic299/1 -> Data Type Conversion720/1
  Shift Arithmetic295/1 -> Data Type Conversion718/1
  Shift Arithmetic291/1 -> Data Type Conversion707/1
  Shift Arithmetic288/1 -> Data Type Conversion702/1
  Bitwise AND403/1 -> Shift Arithmetic287/1
  Shift Arithmetic286/1 -> Data Type Conversion703/1
  Bitwise AND400/1 -> Data Type Conversion701/1
  Demux10/6 -> Data Type Conversion724/1
  Data Type Conversion699/1 -> Bitwise AND400/1, Bitwise AND403/1, Bitwise AND402/1, Bitwise AND401/1
  Bitwise AND402/1 -> Shift Arithmetic286/1
  Bitwise AND425/1 -> Shift Arithmetic306/1
  Shift Arithmetic287/1 -> Data Type Conversion700/1
  Shift Arithmetic306/1 -> Data Type Conversion732/1
  Demux10/2 -> Data Type Conversion704/1
  Bitwise AND401/1 -> Shift Arithmetic288/1
  Data Type Conversion728/1 -> Mux3/95
  Data Type Conversion701/1 -> Mux3/73
  VOUTP_RESSTIMESOCOFFRNGL_s/1 -> Demux10/1
  convert_in24/1 -> Data Type Conversion739/1
  Data Type Conversion739/1 -> Mux3/105
  VOUTP_MAXBATTEMPL_C/1 -> convert_in24/1
  VOUTP_MINBATTEMPL_C/1 -> convert_in25/1
  Data Type Conversion740/1 -> Mux3/106
  convert_in25/1 -> Data Type Conversion740/1
  Bitwise AND434/1 -> Shift Arithmetic310/1
  VOUTP_AVGBATTEMPL_sec/1 -> Data Type Conversion741/1
  Bitwise AND435/1 -> Shift Arithmetic311/1
  Shift Arithmetic312/1 -> Data Type Conversion744/1
  Shift Arithmetic310/1 -> Data Type Conversion745/1
  Data Type Conversion741/1 -> Bitwise AND432/1, Bitwise AND435/1, Bitwise AND434/1, Bitwise AND433/1
  Shift Arithmetic311/1 -> Data Type Conversion742/1
  Bitwise AND433/1 -> Shift Arithmetic312/1
  Bitwise AND432/1 -> Data Type Conversion743/1
  Data Type Conversion742/1 -> Mux3/110
  Data Type Conversion744/1 -> Mux3/108
  Data Type Conversion743/1 -> Mux3/107
  Data Type Conversion745/1 -> Mux3/109
  VOUTP_AVGBATTEMPL_C/1 -> convert_in26/1
  convert_in26/1 -> Data Type Conversion746/1
  Data Type Conversion746/1 -> Mux3/111
  Data Type Conversion751/1 -> Mux3/114
  Data Type Conversion749/1 -> Mux3/112
  Data Type Conversion750/1 -> Mux3/113
  Data Type Conversion748/1 -> Mux3/115
  Bitwise AND436/1 -> Data Type Conversion749/1
  Bitwise AND437/1 -> Shift Arithmetic315/1
  Shift Arithmetic314/1 -> Data Type Conversion748/1
  Data Type Conversion747/1 -> Bitwise AND437/1, Bitwise AND438/1, Bitwise AND439/1, Bitwise AND436/1
  Shift Arithmetic313/1 -> Data Type Conversion751/1
  Shift Arithmetic315/1 -> Data Type Conversion750/1
  Bitwise AND439/1 -> Shift Arithmetic314/1
  VOUTP_BattTempPSAR_sec/1 -> Data Type Conversion747/1
  Bitwise AND438/1 -> Shift Arithmetic313/1
  Bitwise AND442/1 -> Shift Arithmetic316/1
  VOUTP_BattTempPSAL_sec/1 -> Data Type Conversion752/1
  Bitwise AND443/1 -> Shift Arithmetic317/1
  Shift Arithmetic318/1 -> Data Type Conversion755/1
  Shift Arithmetic316/1 -> Data Type Conversion756/1
  Data Type Conversion752/1 -> Bitwise AND440/1, Bitwise AND443/1, Bitwise AND442/1, Bitwise AND441/1
  Shift Arithmetic317/1 -> Data Type Conversion753/1
  Bitwise AND441/1 -> Shift Arithmetic318/1
  Bitwise AND440/1 -> Data Type Conversion754/1
  Data Type Conversion753/1 -> Mux3/119
  Data Type Conversion755/1 -> Mux3/117
  Data Type Conversion754/1 -> Mux3/116
  Data Type Conversion756/1 -> Mux3/118
  Data Type Conversion766/1 -> Mux3/126
  Data Type Conversion764/1 -> Mux3/124
  Data Type Conversion765/1 -> Mux3/125
  Data Type Conversion763/1 -> Mux3/127
  Bitwise AND448/1 -> Data Type Conversion764/1
  Bitwise AND449/1 -> Shift Arithmetic324/1
  Shift Arithmetic323/1 -> Data Type Conversion763/1
  Data Type Conversion762/1 -> Bitwise AND449/1, Bitwise AND450/1, Bitwise AND451/1, Bitwise AND448/1
  Shift Arithmetic322/1 -> Data Type Conversion766/1
  Shift Arithmetic324/1 -> Data Type Conversion765/1
  Bitwise AND451/1 -> Shift Arithmetic323/1
  VOUTP_OVCL_sec/1 -> Data Type Conversion762/1
  Bitwise AND450/1 -> Shift Arithmetic322/1
  Bitwise AND446/1 -> Shift Arithmetic319/1
  VOUTP_OVCR_sec/1 -> Data Type Conversion757/1
  Bitwise AND447/1 -> Shift Arithmetic320/1
  Shift Arithmetic321/1 -> Data Type Conversion760/1
  Shift Arithmetic319/1 -> Data Type Conversion761/1
  Data Type Conversion757/1 -> Bitwise AND444/1, Bitwise AND447/1, Bitwise AND446/1, Bitwise AND445/1
  Shift Arithmetic320/1 -> Data Type Conversion758/1
  Bitwise AND445/1 -> Shift Arithmetic321/1
  Bitwise AND444/1 -> Data Type Conversion759/1
  Data Type Conversion758/1 -> Mux3/123
  Data Type Conversion760/1 -> Mux3/121
  Data Type Conversion759/1 -> Mux3/120
  Data Type Conversion761/1 -> Mux3/122
  Data Type Conversion776/1 -> Mux3/134
  Data Type Conversion774/1 -> Mux3/132
  Data Type Conversion775/1 -> Mux3/133
  Data Type Conversion773/1 -> Mux3/135
  Bitwise AND456/1 -> Data Type Conversion774/1
  Bitwise AND457/1 -> Shift Arithmetic330/1
  Shift Arithmetic329/1 -> Data Type Conversion773/1
  Data Type Conversion772/1 -> Bitwise AND457/1, Bitwise AND458/1, Bitwise AND459/1, Bitwise AND456/1
  Shift Arithmetic328/1 -> Data Type Conversion776/1
  Shift Arithmetic330/1 -> Data Type Conversion775/1
  Bitwise AND459/1 -> Shift Arithmetic329/1
  VOUTP_OFFL_sec/1 -> Data Type Conversion772/1
  Bitwise AND458/1 -> Shift Arithmetic328/1
  Bitwise AND454/1 -> Shift Arithmetic325/1
  VOUTP_OFFR_sec/1 -> Data Type Conversion767/1
  Bitwise AND455/1 -> Shift Arithmetic326/1
  Shift Arithmetic327/1 -> Data Type Conversion770/1
  Shift Arithmetic325/1 -> Data Type Conversion771/1
  Data Type Conversion767/1 -> Bitwise AND452/1, Bitwise AND455/1, Bitwise AND454/1, Bitwise AND453/1
  Shift Arithmetic326/1 -> Data Type Conversion768/1
  Bitwise AND453/1 -> Shift Arithmetic327/1
  Bitwise AND452/1 -> Data Type Conversion769/1
  Data Type Conversion768/1 -> Mux3/131
  Data Type Conversion770/1 -> Mux3/129
  Data Type Conversion769/1 -> Mux3/128
  Data Type Conversion771/1 -> Mux3/130
  Ground_14/1 -> Mux3/149
  Ground_15/1 -> Mux3/150
  Ground_16/1 -> Mux3/151
  Ground_17/1 -> Mux3/152
  Ground_18/1 -> Mux3/153
  Ground_19/1 -> Mux3/154
  Ground_20/1 -> Mux3/155
  Ground_21/1 -> Mux3/156
  Ground_22/1 -> Mux3/157
  Ground_23/1 -> Mux3/158
  Ground_24/1 -> Mux3/159
  Ground_25/1 -> Mux3/160
  Ground_26/1 -> Mux3/161
  Ground_27/1 -> Mux3/162
  Ground_28/1 -> Mux3/163
  Ground_29/1 -> Mux3/164
  Ground_30/1 -> Mux3/165
  Ground_31/1 -> Mux3/166
  Ground_32/1 -> Mux3/167
  Ground_33/1 -> Mux3/168
  Ground_34/1 -> Mux3/169
  Ground_35/1 -> Mux3/170
  Ground_36/1 -> Mux3/171
  Ground_37/1 -> Mux3/172
  Ground_38/1 -> Mux3/173
  Ground_39/1 -> Mux3/174
  Ground_40/1 -> Mux3/175
  Ground_41/1 -> Mux3/176
  Ground_42/1 -> Mux3/177
  Ground_43/1 -> Mux3/178
  Ground_44/1 -> Mux3/179
  Ground_45/1 -> Mux3/180
  Ground_46/1 -> Mux3/181
  Ground_47/1 -> Mux3/182
  Ground_48/1 -> Mux3/183
  Ground_49/1 -> Mux3/184
  Ground_50/1 -> Mux3/185
  Ground_51/1 -> Mux3/186
  Ground_52/1 -> Mux3/187
  Ground_53/1 -> Mux3/188
  Ground_54/1 -> Mux3/189
  Ground_55/1 -> Mux3/190
  Ground_56/1 -> Mux3/191
  Ground_57/1 -> Mux3/192
  Ground_58/1 -> Mux3/193
  Ground_59/1 -> Mux3/194
  Ground_60/1 -> Mux3/195
  Ground_61/1 -> Mux3/196
  Ground_62/1 -> Mux3/197
  Ground_63/1 -> Mux3/198
  Ground_64/1 -> Mux3/199
  Ground_65/1 -> Mux3/200
  Ground_66/1 -> Mux3/201
  Ground_67/1 -> Mux3/202
  Ground_68/1 -> Mux3/203
  Ground_69/1 -> Mux3/204
  Ground_70/1 -> Mux3/205
  Ground_71/1 -> Mux3/206
  Ground_72/1 -> Mux3/207
  Ground_73/1 -> Mux3/208
  Ground_74/1 -> Mux3/209
  Ground_75/1 -> Mux3/210
  Ground_76/1 -> Mux3/211
  Ground_77/1 -> Mux3/212
  Ground_78/1 -> Mux3/213
  Ground_79/1 -> Mux3/214
  Ground_80/1 -> Mux3/215
  Ground_81/1 -> Mux3/216
  Ground_82/1 -> Mux3/217
  Ground_83/1 -> Mux3/218
  Ground_84/1 -> Mux3/219
  Ground_85/1 -> Mux3/220
  Ground_86/1 -> Mux3/221
  Ground_87/1 -> Mux3/222
  Ground_88/1 -> Mux3/223
  Ground_89/1 -> Mux3/224
  Ground_90/1 -> Mux3/225
  Ground_91/1 -> Mux3/226
  Ground_92/1 -> Mux3/227
  Ground_93/1 -> Mux3/228
  Ground_94/1 -> Mux3/229
  Ground_95/1 -> Mux3/230
  Ground_96/1 -> Mux3/231
  Ground_97/1 -> Mux3/232
  Ground_98/1 -> Mux3/233
  Ground_99/1 -> Mux3/234
  Ground_100/1 -> Mux3/235
  Ground_101/1 -> Mux3/236
  Ground_102/1 -> Mux3/237
  Ground_103/1 -> Mux3/238
  Ground_104/1 -> Mux3/239
  Ground_105/1 -> Mux3/240
  Ground_106/1 -> Mux3/241
  Ground_107/1 -> Mux3/242
  Ground_108/1 -> Mux3/243
  Ground_109/1 -> Mux3/244
  Ground_110/1 -> Mux3/245
  Ground_111/1 -> Mux3/246
  Ground_112/1 -> Mux3/247
  Ground_113/1 -> Mux3/248
  Ground_114/1 -> Mux3/249
  Ground_115/1 -> Mux3/250
  Ground_116/1 -> Mux3/251
  Ground_117/1 -> Mux3/252
  Ground_118/1 -> Mux3/253
  Ground_119/1 -> Mux3/254
  Ground_120/1 -> Mux3/255
  Ground_121/1 -> Mux3/256
  VOUTP_HMIKey4FuncSta_enum/1 -> Data Type Conversion782/1
  VOUTP_HMIKey8FuncSta_enum/1 -> Data Type Conversion786/1
  VOUTP_AutoWipHSpdENSta_flg/1 -> Data Type Conversion787/1
  VOUTP_HMIKey3FuncSta_enum/1 -> Data Type Conversion781/1
  VOUTP_HMIKey6FuncSta_enum/1 -> Data Type Conversion784/1
  VOUTP_HMIKey1FuncSta_enum/1 -> Data Type Conversion779/1
  VOUTP_HMIKey5FuncSta_enum/1 -> Data Type Conversion783/1
  VOUTP_HMIKey2FuncSta_enum/1 -> Data Type Conversion780/1
  VOUTP_HMIKey7FuncSta_enum/1 -> Data Type Conversion785/1
  Data Type Conversion779/1 -> Mux3/136
  Data Type Conversion780/1 -> Mux3/137
  Data Type Conversion781/1 -> Mux3/138
  Data Type Conversion782/1 -> Mux3/139
  Data Type Conversion783/1 -> Mux3/140
  Data Type Conversion784/1 -> Mux3/141
  Data Type Conversion785/1 -> Mux3/142
  Data Type Conversion786/1 -> Mux3/143
  Data Type Conversion787/1 -> Mux3/144
  VOUTP_ModelVersionChksum_raw/1 -> Data Type Conversion778/1
  VOUTP_ModelVersion_raw/1 -> Data Type Conversion777/1
  Data Type Conversion777/1 -> Mux3/145
  Data Type Conversion778/1 -> Mux3/146
  VOUTP_DIDModelVersion_raw/1 -> Data Type Conversion788/1
  VOUTP_DIDModelVersionChksum_raw/1 -> Data Type Conversion789/1
  Data Type Conversion788/1 -> Mux3/147
  Data Type Conversion789/1 -> Mux3/148
